simulink model "RB_KAIROS_BaseOnly"  (R2020b)
settings: Solver=ode4  StartTime=0.0  StopTime=t_end  FixedStep=Ts  RelTol=1e-3
values from neighbouring files (symbols this model uses):
  am = 0.3    [RB_KAIROS_ImpControl_OpSpace_BaseOnly.m]
  am_r = 0.3    [RB_KAIROS_ImpControl_OpSpace_BaseOnly.m]
  Jv = [1 0 0; 0 1 0; 0 0 0; 0 0 0; 0 0 0; 0 0 1;]    [RB_KAIROS_ImpControl_OpSpace_BaseOnly.m]
  Kc = diag(5*[1000,1000,0,0,0,1000])    [RB_KAIROS_ImpControl_OpSpace_BaseOnly.m]
  model_sample_time = 0.001    [RB_KAIROS_ImpControl_OpSpace_BaseOnly.m]
  q_dot_0 = zeros(10,1)    [RB_KAIROS_ImpControl_OpSpace_BaseOnly.m]
  T_i = T_W_V    [RB_KAIROS_ImpControl_OpSpace_BaseOnly.m]
  tau_ext = [0 0 0]    [RB_KAIROS_ImpControl_OpSpace_BaseOnly.m]
  v_SMU = 10    [RB_KAIROS_ImpControl_OpSpace_BaseOnly.m]
  vm = 0.6    [RB_KAIROS_ImpControl_OpSpace_BaseOnly.m]
  vm_r = 0.6    [RB_KAIROS_ImpControl_OpSpace_BaseOnly.m]
undefined symbols (not defined in the file or in its folder): DiscIntNeverNeededParam, magnitude, q_0, T_f
libraries: simulink x4, utils x4, transformations_lib x1
(part 15 of 16)

== matlab function RB_KAIROS_BaseOnly/Trajectory Generator/move2pose/Cartesian_ipol2/translation/Embedded MATLAB Function1 ==
  data: t input; qd output; s0 input; v0 input; sf input; vd input; am input; Tm input; T_scale input; interpoly input; time_step input; start_opt input; rethink_point input; start_lvl input; stop_lvl input; v_smu input; vm input; dqd output; ddqd output; ipol_finished output; opti_break output; T_est output
function [qd,dqd,ddqd, ipol_finished, opti_break, T_est] = calc_qd(t,s0,v0,sf,vd,am,Tm,T_scale,interpoly,time_step,start_opt,rethink_point,start_lvl,stop_lvl,v_smu,vm)
%%% This function decides which version to call; Or when/if a rethink is
%%% done.
% 0 = internship version (only with minor bugfixes)
% 1 = start with half the velocity, then rethink, then linear part and
% rest is the original full half
% 2 = start with full half rethink, again full half (Mazins way)
% 3 = general solution, heading to vm always (best option)
% 4 = general solution, heading to v_smu if going down (Mazins way)

qd = 0;
dqd = 0;
ddqd = 0;
ipol_finished = 0;
opti_break = 0;
T_est = 0;
switch rethink_point
    case 0
        [qd,dqd,ddqd, ipol_finished] = calc_qd_f(t,s0,v0,sf,vd,am,T_scale,interpoly,time_step);
    case 1
        [qd,dqd,ddqd, ipol_finished, opti_break, T_est] = calc_qd_hlf(t,s0,v0,sf,vd,am,Tm,T_scale,interpoly,time_step,start_opt);
    case 2
        [qd,dqd,ddqd, ipol_finished, opti_break, T_est] = calc_qd_ff(t,s0,v0,sf,vd,am,Tm,T_scale,interpoly,time_step,start_opt);
    case 3
        [qd,dqd,ddqd, ipol_finished, opti_break, T_est] = calc_qd_g(t,s0,v0,sf,vd,am,Tm,T_scale,interpoly,time_step,start_opt,start_lvl,stop_lvl,v_smu,vm,rethink_point);
    case 4
        [qd,dqd,ddqd, ipol_finished, opti_break, T_est] = calc_qd_g(t,s0,v0,sf,vd,am,Tm,T_scale,interpoly,time_step,start_opt,start_lvl,stop_lvl,v_smu,vm,rethink_point);
    otherwise
        error('Unknown rethink_point');       %rest
end


end

function [qd,dqd,ddqd, ipol_finished, opti_break, T_est] = calc_qd_g(t,s0,v0,sf,vd,am,Tm,T_scale,interpoly,time_step,start_opt,start_lvl,stop_lvl,v_smu,vm,rethink_point)
% This function calculates a one dimensional movement with a trapezodial 
% signal for velocity over time. Additionally it is able to adapt to shifts
% in the maximum allowed velocity.
%
% This is the most general solution so far. It accelerates till am and then
% it stays on this level till it has to decelerate again to reach the new
% velocity level. The velocity level could be updated in any timestep.
%
% Inputs:
% t         current runtime
% s0        start value for motion in position
% v0        start value for motion in velocity
% sf        final value for motion in position
% vd        desired velocity
% am        maximum allowed acceleration
% Tm        Maximum time left for adaption
% T_scale   Scaling factor for duration of adaption
% interpoly Which interpolation to use
% time_step Duration of one time step
% start_opt Options for prevent errors at start and end; see below
% start_lvl percentage for delta_v_start: [0;1[ (Do not set to near to one!)
% stop_lvl  percentage for delta_v_stop: [0;1[ (Do not set to near to one!)
% v_smu     Real v_smu
% vm        maximum allowed velocity
% rethink_point
%           choose on which velocity the percentage is used
%
% Outputs:
% qd        disered position at current time
% dqd       disered velocity at current time
% ddqd      disered acceleration at current time
% ipol_finished 
%           motion is finished
% opti_break
%           Trigger for optimal breaking; is set to 1 if Tm<T_est
% T_est     Current estimate of the duration of the adaption motion

% Start / end options:
% 0 = Do nothing; Not recommanded, because of unstable behaviour, since start phase not programmed
% 1 = Delay till adaption possible (Best option I think)
% 2 = Delay till adaption possible and vd is updated


% In general variables with ..._1 belong to previous runs of the code and
% variables with numbers at the end belong to the corresponding phase. 
% Phase 1 is the start of an adaption motion. On this phase the
% acceleration is increased to am. In phase 2 the acceleration is constant
% on level am, which means that the velocity is linear. The decrease of the
% acceleration to zero again is called phase 3.
% A single i in the name of a varibale, means an inital value of something
% and the same holds for f for final value. m is maximum, d is desired, c
% is current.
% q is a vector with (position,velocity,acceleration). Small t is a absolut
% time, whereas capital T is a time duration.


T_est = 0; %init Duration estimate
v_eps = 1e-4; %lowest velocity difference an adaption starts

% Code can not stop the motion => vd must be >0 (because of t_shift calc)
if vd<v_eps
    vd=v_eps;
end

%% Initialize persistent variables for adaption motion
persistent vd_1 adpt adpt_run phase restart ti1 qi1 qf1 T1 t_shift t_shift3 t_shift_1 T2 T3 ti2 parameter2 ti3 qf3 qi3 delta_q3 adpt_blanking adpt_blanking_end opti_break_mem v_delta_stop v_delta_start
if isempty(vd_1)
    vd_1 = vd;       %remembers the max velocity from last run
end
if isempty(adpt)
    adpt = false;   %stores if an adaption motion is activated
end
if isempty(adpt_run)
    adpt_run = false;   %stores if an adaption motion is activated
end
if isempty(phase)
    phase = 0;         %phase of adaption
end
if isempty(restart)
    restart = -1;         %At end of phase 3 the current velocity must be stored and restarts an adpation process
end
if isempty(t_shift)
    t_shift = 0;    %Time distance with which the current reference motion is shifted
end
if isempty(t_shift_1)
    t_shift_1 = 0;    %Time distance with which the old reference motion was shifted
end
if isempty(ti1)
    ti1 = 0;         %Initial time step for adaption motion
end
if isempty(T1)
    T1 = 0;          %Duration of complete adaption motion; tf = ti+T
end
if isempty(qi1)
    qi1 = zeros(3,1);%Initial values (pos,vel,acc) for adaption motion
end
if isempty(qf1)
    qf1 = zeros(3,1);%Final values (pos,vel,acc) for adaption motion
end
if isempty(ti2) 
    ti2 = 0;         %Initial time for linear part  (phase 2)
end
if isempty(T2)
    T2 = 0;         %Exact duration of phase 2
end
if isempty(parameter2)
    parameter2 = zeros(3,1);         %Parameter of linear part / phase 2: 0.5*p(3)*t^2 + p(2)*t + p(1)
end
if isempty(ti3)
    ti3 = 0;         %Initial time for phase 3
end
if isempty(T3)
    T3 = 0;         %Duration of phase 3 (But seen from start in the past; so actually it is T/2)
end
if isempty(qi3)
    qi3 = zeros(3,1); %Initial values (pos,vel,acc) for phase 3
end
if isempty(qf3)
    qf3 = zeros(3,1); %Final values (pos,vel,acc) for phase 3
end
if isempty(t_shift3)
    t_shift3 = 0;    %Time distance with which the updated reference motion is shifted (phase 3)
end
if isempty(delta_q3)
    delta_q3 = 0;         %shift of position in phase 3
end
if isempty(adpt_blanking)
    adpt_blanking = -1;         %memory of current vd for startopt 2
end
if isempty(adpt_blanking_end)
    adpt_blanking_end = -1;         %memory of last vd before adaption while deceleration phase
end
if isempty(opti_break_mem)
    opti_break_mem = 0;         %memory of opti break; (holds trigger while adaption)
end
if isempty(v_delta_start)
    v_delta_start = 0;         %delta of velocity which the start of an adaption needs
end
if isempty(v_delta_stop)
    v_delta_stop = 0;         %delta of velocity which the stop of an adaption needs
end

%% This If runs only for one timestep!!!
% If current desired velocity is unequal to old one 
% Not directly at the beginning
% Dont start new while a adaption is still running, to prevent reset of
%   initial values
% Or restart is requested at end of last adaption
% And do nothing anymore if last adaption has collided with end 
if adpt_blanking_end==-1 && adpt==false && (...
        (vd~=vd_1 && t>time_step)...
        || restart>=0 )
            
    
    if restart==vd %This if prevents a adaption if restart was set to the current vd (only possible with startoptions or low velocity)
        adpt = false;
        phase = 0;
        restart = -1;
        adpt_blanking = -1;
        
    % This if prevents adaptions if the difference in the desired velocity
    % is below the threshold v_eps. To save the current velocity the
    % restart variable is used again. This also means that if the vd is
    % changing with a rate lower than the threshold, it is neccessary to
    % also compare the current velocity (in restart) and the current
    % desired velocity. If these two are more than the threshold it is
    % possible to adapt with the minimum adaption function.
    elseif (restart==-1 && abs(vd-vd_1)<v_eps) ||...
           (restart>=0  && abs(vd-vd_1)<v_eps && abs(vd-restart)<v_eps)
        adpt = false; 
        phase = 0;
        if restart == -1 %For preventing a small error, because the vd has changed, while the non-adaption calculation
           restart = vd_1; 
        end
        
    % If no reasons so far to prevent adaption, start the adaption:
    else
        adpt = true;          % Activate adaption 
        phase = 1;            % Start with phase 1
        t_shift_1 = t_shift;  % Store old time shift if adaption is reseted because of start/end phase of mogen 
        ti1 = t;              % Set initial timestep to current step  

        %%% inital set of position, velo, acceleration for adaption motion 
        % is the same as the old mogen would do (t_shift is not updated at
        % this time!)
        if restart>=0 %If restart is requested, the current velocity is stored in the restart variable
            [qi1, ~] = interpolator(ti1+t_shift, compute_traj_parameters(s0, v0, sf, restart, am));
        else
            [qi1, ~] = interpolator(ti1+t_shift, compute_traj_parameters(s0, v0, sf, vd_1, am));
        end

        %%% Calc basic velocity levels
        vc = qi1(2);    % current velocity = restart velocity or vd_1
        vf = vd;        % v_final is current global final velocity
        v_heading = vf; % v_heading the velocity level the program is looking to, while calculating the v_deltas

        %For making sure that it is heading to v_smu always, while going down (Mazins way)
        if rethink_point == 4 && vd<vc
            v_heading = v_smu; 
        end

        % velocity deltas at begin and end of adaption: 
        % mind the signs!!
        v_delta_start = ((v_heading-vc)*(1-start_lvl))/2;
        v_delta_stop  = ((vc-v_heading)*(1-stop_lvl))/2;

        %%% Calculation of Phase 1 and basic parameters

        % computes the time shift for shifting the new motion to the end
        % point of the old motion. So at which time the new motion has
        % the same qd? Then calculate the time distance to the inital
        % time of the change in velocities
        % t_shift < 0 if new motion is faster (vd>vd_1)
        % t_shift > 0 if new motion is slower (vd<vd_1)
        % interpolator_1 is the inverse function of interpolator!
        vf1 = vc+2*v_delta_start; %This is the final velocity of the start / phase 1
        t_shift_inv = interpolator_1(qi1(1), compute_traj_parameters(s0, v0, sf, vf1, am));
        t_shift = t_shift_inv - ti1 ;

        % Calculate duration of adaption in phase 1
        if interpoly==0 % if interpolation is zero no adaption is requested, but the t_shift has to be calculated anyway
            adpt = false;
            phase = 0;
            restart = -1;
            adpt_blanking = -1;
        else
            T1 = T_calc(vc,vf1,am,T_scale,interpoly); 
            %T1 = T_calc_a_scale(vc,vf1,vm,v_eps,am,time_step,T_scale,interpoly); 
        end

        % The additional shift for adaption motion is dependent on the
        % difference in the velocities. See report for details.
        t_shift = t_shift+(T1/2)*((vc/vf1)-1);

        % Calculate final values for adaption motion. Which are reached
        % at inital time plus duration of adaption and new time shift
        [qf1, ~] = interpolator(ti1+t_shift+T1, compute_traj_parameters(s0, v0, sf, vf1, am));

        %%% Parameters for Phase 2 / linear part

        ti2 = ti1+T1/2; % initial time of linear part

        % calculate state of phase 1 at start of phase 2, which are the
        % parameters of phase 2, since phase 2 has its time orgin at the
        % same point.
        parameter2 = adpt_fct(ti2,ti1,T1,qi1,qf1,vd,am,interpoly); 

        %%% Check if errors occured so far due to acc/dec phase
        % check start phase
        if qi1(3)>0 || qf1(3)>0 || t_shift_inv == 0 %If interpolator in acc phase or invers interpolator is not jet available
            if start_opt == 1 
                adpt = false; 
                phase = 0;
                t_shift = t_shift_1; %Reset calculated t_shift
                if restart == -1 % For delaying the start of the adaption, the restart is used and set to the current value, if not done already
                   restart = vd_1; 
                end
            elseif start_opt == 2 % For delay and wait on update, the restart is set and ...
                adpt = false;
                phase = 0;
                t_shift = t_shift_1; %Reset calculated t_shift
                adpt_blanking = vd; % ... the adpt_blanking variable is set to the current new velocity.
                if restart == -1
                   restart = vd_1; 
                end
            end
        elseif start_opt>0 && (qi1(3)<0 || qf1(3)<0 || t_shift_inv == -1 ) %If interpolator in dec phase or invers interpolator is no more available
            % if adaption is colliding with the decelaration phase of mogen,
            % the adpt_blanking_end variable is used, which prevents all
            % atempts for an adaption
            if restart>=0
                adpt_blanking_end = restart; %If the adaption was triggerd with restart, the current velocity is there too
            else
                adpt_blanking_end = vd_1;
            end
            adpt = false; 
            phase = 0;
            t_shift = t_shift_1;
            restart = -1;
            adpt_blanking = -1;
        elseif adpt_blanking == vd % Only for startopt==2: If adaption would be possible, the code now waites for an update of vd.
            adpt = false;
            phase = 0;
            t_shift = t_shift_1;
        end  
    end
end

%% Update function; runs always in phase 1 and phase 2 to update duration and check final levels
if adpt == true && (phase == 1 || phase == 2)
    
    %%% First decide to which velocity the program should go. This is
    %%% necessesary since the current vd could be higher than the velocity
    %%% level wich could be reached with an imdiate introduction of phase
    %%% 3. This nearest velocity level which can currently be reached is
    %%% called v_near and calculated first   
    
    % evaluate linear part at last timestep
    t2 = t-ti2-time_step; 
    q2 = zeros(3,1); 
    q2(1) = 0.5*parameter2(3)*t2^2+parameter2(2)*t2+parameter2(1);
    q2(2) = parameter2(3)*t2+parameter2(2);
    q2(3) = parameter2(3);

    % Calculate nearest velocity v_near
    if phase == 1
        % in phase 1 it is the start velocity plus both deltas, without
        % linear part
        v_near = qi1(2)+v_delta_start-v_delta_stop; %mind the signs!!!
    else
        % while linear part it is the current velocity level plus what is
        % needed to stop adaption.
        v_near = q2(2)-v_delta_stop; %mind the signs!!!
    end
    
    % this is now the decision to which velocity the update should go to
    if qi1(2)>qf1(2) && vd>=v_near
        vd_up = v_near;
    elseif qi1(2)<qf1(2) && vd<=v_near
        vd_up = v_near;
    else
        % check if it is still possible to reach at least v_near in the
        % next step (called v_near_p1). Because if the vd changes in the
        % next step so that it is no more possible to reach vd, the
        % adaption has to stop at v_near_p1 in the next step and therefore
        % v_near_p1 has to be reachable. If even this is not possible, then
        % stop now at v_near.

        % evaluate linear part at current timestep
        t2 = t-ti2; 
        q2 = zeros(3,1); 
        q2(1) = 0.5*parameter2(3)*t2^2+parameter2(2)*t2+parameter2(1);
        q2(2) = parameter2(3)*t2+parameter2(2);
        q2(3) = parameter2(3);

        % Calculate nearest velocity v_near_p1
        if phase == 1
            % in phase 1 it is the start velocity plus both deltas, without
            % linear part
            v_near_p1 = qi1(2)+v_delta_start-v_delta_stop; %mind the signs!!!
        else
            % while linear part it is the current velocity level plus what is
            % needed to stop adaption.
            v_near_p1 = q2(2)-v_delta_stop; %mind the signs!!!
        end
        
        % Evaluate function at v_near_p1 for next time step
        [~,~,~,~,~,~,~,error_state_p1] = calc_g_update_fct(v_near_p1,v_delta_stop,qi1,ti2,parameter2,am,T_scale,interpoly,s0, v0, sf,start_opt,vm,v_eps,time_step);
        if start_opt >0 && error_state_p1==2 %If errors with dec phase
            vd_up = v_near;
        else        
            vd_up = vd;
        end
    end 
    
    [T2,T3,ti3,qi3,qf3,delta_q3,t_shift3,error_state] = calc_g_update_fct(vd_up,v_delta_stop,qi1,ti2,parameter2,am,T_scale,interpoly,s0, v0, sf,start_opt,vm,v_eps,time_step);
    
    if adpt_run==false
        %%% Check if adaption is possible before it actually has started; means check error_state
        if error_state==1 %If errors with acc phase
            if start_opt == 1 
                adpt = false; 
                phase = 0;
                t_shift = t_shift_1; %Reset calculated t_shift
                if restart == -1 % For delaying the start of the adaption, the restart is used and set to the current value, if not done already
                   restart = vd_1; 
                end
            elseif start_opt == 2 % For delay and wait on update, the restart is set and ...
                adpt = false;
                phase = 0;
                t_shift = t_shift_1; %Reset calculated t_shift
                adpt_blanking = vd; % ... the adpt_blanking variable is set to the current new velocity.
                if restart == -1
                   restart = vd_1; 
                end
            end
        elseif start_opt >0 && error_state==2 %If errors with dec phase
            % if adaption is colliding with the decelaration phase of mogen,
            % the adpt_blanking_end variable is used, which prevents all
            % atempts for an adaption
            if restart>=0
                adpt_blanking_end = restart; %If the adaption was triggerd with restart, the current velocity is there too
            else
                adpt_blanking_end = vd_1;
            end
            adpt = false; 
            phase = 0;
            t_shift = t_shift_1;
            restart = -1;
            adpt_blanking = -1;
        else % Triggered if adaption is possible and will start now
            % Reset variables
            restart = -1;
            adpt_blanking = -1;
        end 
    else
        % adaption is already running; means no problems possible at start 
        % points, but if current endpoint is colliding with deceleration
        % phase, take v_near to stop.
        if start_opt >0 && error_state==2 %If errors with dec phase
            [T2,T3,ti3,qi3,qf3,delta_q3,t_shift3,~] = calc_g_update_fct(v_near,v_delta_stop,qi1,ti2,parameter2,am,T_scale,interpoly,s0, v0, sf,start_opt,vm,v_eps,time_step);
        end
    end

end

%% This If runs only for one timestep!!!
% Phase 1 => Phase 2
if phase == 1 && t>=ti2 %End of phase 1
    phase = 2;
end

%% This If runs only for one timestep!!!
% Phase 2 => Phase 3
if phase == 2 && t>=ti3 %End of phase 2
    phase = 3;
    t_shift = t_shift3; %Activate new t_shift for phase 3
end

%% Here the actual motion is calculated
% Interpolates the values of pos,vel,acc (qv) with parameters and current time t 

if restart >=0
    [qdv, ipol_finished] = interpolator(t+t_shift, compute_traj_parameters(s0, v0, sf, restart, am));
elseif adpt_blanking_end >=0
    [qdv, ipol_finished] = interpolator(t+t_shift, compute_traj_parameters(s0, v0, sf, adpt_blanking_end, am));
else
    [qdv, ipol_finished] = interpolator(t+t_shift, compute_traj_parameters(s0, v0, sf, vd, am));
end  

%% If adaption motion needed
if adpt == true
    
    adpt_run = true;
    ipol_finished=0;%Prevent finish command from old interpolator
    % Calc adaption motion
    if phase == 1
        % opti_break
        T_est = (T1/2+T2+T3/2)-(t-ti1);
        if Tm<T_est
            opti_break_mem = 1; 
        end
        % accelerate till am
        qdv = adpt_fct(t,ti1,T1,qi1,qf1,vd,am,interpoly);
    elseif phase == 2
        % opti_break
        T_est = ((T2+T3/2)-(t-ti2));
        if Tm<T_est
            opti_break_mem = 1; 
        end
        % linear part
        t2 = t-ti2;
        qdv = zeros(3,1);
        qdv(1) = 0.5*parameter2(3)*t2^2+parameter2(2)*t2+parameter2(1);
        qdv(2) = parameter2(3)*t2+parameter2(2);
        qdv(3) = parameter2(3);
    elseif phase == 3
        %if time is equal than the finish time => adaption motion is complete
        %But it is aborted one timestep earlier, since the finish timestep
        %is already computed correctly by the standard interpolator.
        if t>=ti3+T3/2-1*time_step  
            adpt=false;     %If adaption finished => reset
            phase = 0;
            adpt_run = false;
            opti_break_mem = 0; % also reset opti break
            % Calculate finish time_step here because vd could be not equal
            % to final reached velocity level
            [qdv, ipol_finished] = interpolator(t+t_shift, compute_traj_parameters(s0, v0, sf, qf3(2), am)); 
            if vd~=qf3(2)  %If adaption is finished, but the vd value has changed again => restart from current velocity on
                restart = qf3(2);
            else
                restart = -1;
            end            
        else
            % opti_break
            T_est = T3/2-(t-ti3);
            if Tm<T_est
                opti_break_mem = 1; 
            end
        
            % Adaption to vd velocity
            delta_q_vec = zeros(3,1);
            delta_q_vec(1) = delta_q3; %Build delta_q vector
            tx = -T3/2;
            % Evaluate adaption function, shift with tx in time ...
            qdv = adpt_fct(t,ti3+tx,T3,qi3,qf3,vd,am,interpoly) - delta_q_vec;
        end 
        
    end

end

%% Set output
if sf == s0          % No motion needed if start = end 
    qd = s0;         % => set initial values
    dqd = v0;
    ddqd = 0;  
else     
    qd = qdv(1);     % set output
    dqd = qdv(2);
    ddqd = qdv(3);        
end
opti_break = opti_break_mem; %set opti break output (Simulink cannot use persistent variable as output)
vd_1 = vd;  %remember current max velocity

end

function [qd,dqd,ddqd, ipol_finished, opti_break, T_est] = calc_qd_hlf(t,s0,v0,sf,vm,am,Tm,T_scale,interpoly,time_step,start_opt)
% This function calculates a one dimensional movement with a trapezodial 
% signal for velocity over time. Additionally it is able to adapt to shifts
% in the maximum allowed velocity.
%
% This is the more adaptive version which rethinks about the target
% velocity after the maximum acceleration is reached. And also it is
% allowed to change the velocity reference while an adaption is running.
%
% Inputs:
% t         current runtime
% s0        start value for motion in position
% v0        start value for motion in velocity
% sf        final value for motion in position
% vm        maximum allowed velocity
% am        maximum allowed acceleration
% Tm        Maximum time left for adaption
% T_scale   Scaling factor for duration of adaption
% interpoly Which interpolation to use
% time_step Duration of one time step
% start_opt Options for prevent errors at start and end; see below
%
% Outputs:
% qd        disered position at current time
% dqd       disered velocity at current time
% ddqd      disered acceleration at current time
% ipol_finished 
%           motion is finished
% opti_break
%           Trigger for optimal breaking; is set to 1 if Tm<T_est
% T_est     Current estimate of the duration of the adaption motion

% Start / end options:
% 0 = Do nothing; Not recommanded, because of unstable behaviour, since start phase not programmed
% 1 = Delay till adaption possible (Best option I think)
% 2 = Delay till adaption possible and vm is updated

%% Initialize persistent variables for adaption motion
persistent vm1 adpt phase restart ti qi qf T t_shift t_shift_up t_shift_1 T_lin T_up vf ti_lin shift slope c ti_up qf_up qi_up delta_q adpt_blanking adpt_blanking_end opti_break_mem
if isempty(vm1)
    vm1 = vm;       %remembers the max velocity from last run
end
if isempty(adpt)
    adpt = false;   %stores if an adaption motion is activated
end
if isempty(phase)
    phase = 0;         %phase of adaption
end
if isempty(restart)
    restart = -1;         %At end of phase 4 the current velocity must be stored and restarts an adpation process
end
if isempty(ti)
    ti = 0;         %Initial time step for adaption motion
end
if isempty(qi)
    qi = zeros(3,1);%Initial values (pos,vel,acc) for adaption motion
end
if isempty(qf)
    qf = zeros(3,1);%Final values (pos,vel,acc) for adaption motion
end
if isempty(T)
    T = 0;          %Duration of complete adaption motion; tf = ti+T
end
if isempty(t_shift)
    t_shift = 0;    %Time distance with which the current reference motion is shifted
end
if isempty(t_shift_up)
    t_shift_up = 0;    %Time distance with which the updated reference motion is shifted
end
if isempty(t_shift_1)
    t_shift_1 = 0;    %Time distance with which the old reference motion was shifted
end
if isempty(T_lin)
    T_lin = 0;         %Exact duration of phase 2
end
if isempty(T_up)
    T_up = 0;         %Duration of phase 3 (But seen from start in the past; so actually it is T/2)
end
if isempty(vf)
    vf = 0;         %global final velocity at start of adaption motion
end
if isempty(ti_lin) 
    ti_lin = 0;         %Initial time for linear part  (phase 2)
end
if isempty(shift)
    shift = 0;         %shift of linear part (phase 2)
end
if isempty(slope)
    slope = 0;         %slope of linear part (phase 2)
end
if isempty(c)
    c = 0;         %integration const of linear part (phase 2)
end
if isempty(ti_up)
    ti_up = 0;         %Initial time for phase 3
end
if isempty(qf_up)
    qf_up = zeros(3,1); %Final values (pos,vel,acc) for phase 3
end
if isempty(qi_up)
    qi_up = zeros(3,1); %Initial values (pos,vel,acc) for phase 3
end
if isempty(delta_q)
    delta_q = 0;         %shift of position in phase 3
end
if isempty(adpt_blanking)
    adpt_blanking = -1;         %memory of current vm for startopt 2
end
if isempty(adpt_blanking_end)
    adpt_blanking_end = -1;         %memory of last vm before adaption while deceleration phase
end
if isempty(opti_break_mem)
    opti_break_mem = 0;         %memory of opti break; (holds trigger while adaption)
end
T_est = 0; %init

%% This If runs only for one timestep!!!
% If current max velocity is unequal to old one 
% Not directly at the beginning
% Dont start new while a adaption is still running, to prevent reset of
%   initial values
% Or restart is requested at end of last adaption
if abs(vm-vm1)>1e-3 && t>time_step && adpt==false ...
        || restart>=0 && adpt==false  
    adpt = true;          % Activate adaption         
    ti = t;               % Set initial timestep to current step  
    
    %init some variables for simulink
    t_inv = 0; 
    t_inv_f = 0;
    v_current = 0;
    v_goal = 0;
    
    if restart==vm %This if prevents a adaption if restart was set to the current vm (only with startoptions)
        adpt = false;
        ti = 0;
        restart = -1;
        adpt_blanking = -1;
    else
        %%% inital set of position, velo, acceleration for adaption motion 
        % is the same as the old mogen would do (t_shift is not updated at
        % this time!)
        if restart>=0 %If restart is requested, the current velocity is stored in the restart variable
            [qi, ~] = interpolator(ti+t_shift, compute_traj_parameters(s0, v0, sf, restart, am));
        else
            [qi, ~] = interpolator(ti+t_shift, compute_traj_parameters(s0, v0, sf, vm1, am));
        end

        vf = vm; % vf is current global final velocity
        v_current = qi(2); % current velocity = restart velocity or vm1
        v_goal = 0.5*(vf+v_current); %intermediate goal velocity

        % Check if adaption is possible; Therefore the inverse functions
        % must be available.
        t_inv = interpolator_1(qi(1), compute_traj_parameters(s0, v0, sf, v_goal, am)) ;
        t_inv_f = interpolator_1(qi(1), compute_traj_parameters(s0, v0, sf, vf, am));
        % If they return zero an adaption is not possible since start phase
        % is active; 
        % Another reason for no adaption is that the current acceleration 
        % is not zero.
        if t_inv == 0 || t_inv_f == 0 || qi(3)>0
            if start_opt == 1 % For delaying the start, the restart is used and set to the current value, if not done already
                adpt = false; 
                ti = 0;
                if restart == -1
                   restart = vm1; 
                end
            elseif start_opt == 2 % For delay and wait on update, the restart is set and ...
                adpt = false;
                ti = 0;
                adpt_blanking = vm; % ... the adpt_blanking variable is set to the current new velocity.
                if restart == -1
                   restart = vm1; 
                end
            end
        end  
    end
    
    if start_opt >0 && qi(3)<0
        adpt_blanking_end = vm1;
        adpt = false; 
        ti = 0;
        restart = -1;
        adpt_blanking = -1;
    end
    
    if adpt_blanking == vm % Only for startopt==2: If adaption would be possible, the code now waites for an update of vm.
        adpt = false;
        ti = 0;
    end
    
    if adpt == true
        % Really start with an adaption now!
        phase = 1;            % Start with phase 1

        % Store old time shift for later calculation of virtual shift
        t_shift_1 = t_shift;

        %%% Calculation of Phase 4 and basic parameters
        
        % computes the time shift for shifting the new motion to the end
        % point of the old motion. So at which time the new motion has
        % the same qd? Then calculate the time distance to the inital
        % time of the change in velocities
        % t_shift < 0 if new motion is faster (vm>vm1)
        % t_shift > 0 if new motion is slower (vm<vm1)
        % interpolator_1 is the inverse function of interpolator!
        t_shift = t_inv - ti ;

        % Calculate duration of adaption
        if interpoly==0 
            T = 0;
            adpt = false;
            phase = 0;
        else
            T = T_calc(v_current,v_goal,am,T_scale,interpoly)*2; %*2 to fit to Mazins way
        end

        % The additional shift for adaption motion is dependent on the
        % difference in the velocities. See report for details.
        t_shift = t_shift+(T/4)*((v_current/v_goal)-1);

        % Calculate final values for adaption motion. Which are reached
        % at inital time plus duration of adaption and new time shift
        [qf, ~] = interpolator(ti+t_shift+T/2, compute_traj_parameters(s0, v0, sf, v_goal, am));

        %%% Parameters for Phase 2 / linear part
        
        ti_lin = ti+T/4; % initial time of linear part
        
        % calculate current state with adaption from phase 1
        q_current = adpt_fct(ti_lin,ti,T/2,qi,qf,vm,am,interpoly);        
        
        % Calculate parameters for linear part in phase 2
        slope = q_current(3);   %slope of lin part is acceleration of current state
        shift = q_current(2);   %shift of lin part is velocity of current state
        c = q_current(1);       %Position constant is position of current state
        T_lin = ((0.5*(qi(2)+vf)-shift)/slope);% Exact Duration of linear part

        
        %%% Parameters for Phase 3
        ti_up = ti_lin+T_lin; % initial time for phase 3
    
        % calculate what linear part would do now = final value of phase 2
        dt = T_lin;
        qf_lin = zeros(3,1); %final value of phase 2
        qf_lin(1) = 0.5*slope*dt^2+shift*dt+c;
        qf_lin(2) = slope*dt+shift;
        qf_lin(3) = slope;

        T_up = T; % This not directly the duration of phase 3, because of the virtual part in the past
        qi_up = qi; % The final adaption motion starts at the same point as the first
        tx = (T/4)-T_lin; %exact time shift resulting from linear part

        % Calculate a time shift for the interpolator, as if the vf was
        % triggered right at the start (ti)
        t_shift_inter = t_inv_f - ti ;
        t_shift_inter = t_shift_inter+(T/2)*((qi_up(2)/vf)-1);

        % Also calculate final values, as if the vf was triggered right at the
        % start.
        [qf_up, ~] = interpolator(ti+t_shift_inter+T, compute_traj_parameters(s0, v0, sf, vf, am));

        % From now on this initial and final values are used in the adaption
        % function for the phase 3. This function is now also shifted in time
        % with the tx value, so starting time is ti-tx.

        % Next step is to evaluate this function at ti_up, which is the current
        % time, to get the position is function would do.
        q_dir_adpt = adpt_fct(ti_up,ti-tx,T_up,qi_up,qf_up,vm,am,interpoly);
        % The difference of the adaption motion position and current position
        % of the final values of the linear part, is now used to shift the
        % adaption also in position level to the current values.
        delta_q = q_dir_adpt(1) - qf_lin(1);
        delta_q_vec = zeros(3,1);
        delta_q_vec(1) = delta_q;

        % Next step is to calculate the real final values, which are the same
        % as the direct ones in velocity and acceleration level. But for
        % position level one needs to respect the delta_q shift.
        qf_real = qf_up - delta_q_vec;

        % To fit the interploator function at this final values again, a new
        % time shift is calculated 
        t_shift_up = interpolator_1(qf_real(1), compute_traj_parameters(s0, v0, sf, vf, am)) - (ti+T_up-tx) ;

        % test line; Should be all ==0
        %test_diff = q_dir_adpt-delta_q_vec -qf_lin;

        
        %%% blanking for deceleration phase
        if start_opt >0 && (qf(3)~=0 || qf_up(3)~=0)
            if restart>=0
                adpt_blanking_end = restart;
            else
                adpt_blanking_end = vm1;
            end
            adpt = false;
            phase = 0;
            t_shift = t_shift_1;
        end
        
        % Reset variables
        restart = -1;
        adpt_blanking = -1;
        
    end
end
    
%% This If runs only for one timestep!!!
% Rethink?! Phase 1 => Phase 2
if phase == 1 && t>=ti_lin %End of phase 1
    if qi(2)<vf && vm<=qf(2) % If human stops or goes away meanwhile
        phase = 4;
    elseif qi(2)>vf && vm>=qf(2) % If human stops or goes away meanwhile
        phase = 4;
    else
        phase = 2;
    end 
end

%% This If runs only for one timestep!!!
% Phase 2 => Phase 3
if phase == 2 && t>=ti_up %End of phase 2
    phase = 3;
    t_shift = t_shift_up;
end

%% Here the actual motion is calculated
% Interpolates the values of pos,vel,acc (qv) with parameters and current time t 

if restart >=0
    [qdv, ipol_finished] = interpolator(t+t_shift, compute_traj_parameters(s0, v0, sf, restart, am));
elseif adpt_blanking_end >=0
    [qdv, ipol_finished] = interpolator(t+t_shift, compute_traj_parameters(s0, v0, sf, adpt_blanking_end, am));
else
    [qdv, ipol_finished] = interpolator(t+t_shift, compute_traj_parameters(s0, v0, sf, vm, am));
end  

%% If adaption motion needed
if adpt == true
    
    %%% Calc adaption motion
    ipol_finished=0;%Prevent finish command from old interpolator
    if phase == 1
        %%% opti_break
        T_est = ((0.75*T+T_lin)-(t-ti));
        if Tm<T_est
            opti_break_mem = 1; 
        end
        % accelerate till am
        qdv = adpt_fct(t,ti,T/2,qi,qf,vm,am,interpoly);
    elseif phase == 2
        %%% opti_break
        T_est = ((0.5*T+T_lin)-(t-ti_lin));
        if Tm<T_est
            opti_break_mem = 1; 
        end
        % linear part
        qdv = zeros(3,1);
        dt = t-ti_lin;
        qdv(1) = 0.5*slope*dt^2+shift*dt+c;
        qdv(2) = slope*dt+shift;
        qdv(3) = slope;
    elseif phase == 3
        % decelerate to 0 and reach vf
        
        tx = (T/4)-T_lin; %exact time shift of linear part (again)
        %if time is equal than the finish time => adaption motion is complete
        %But it is aborted one timestep earlier, since the finish timestep
        %is already computed correctly by the standard interpolator.
        if t>=(ti-tx+T_up-1*time_step) 
            adpt=false;     %If adaption finished => reset
            phase = 0;
            opti_break_mem = 0; 
            % Calculate finish time_step
            [qdv, ipol_finished] = interpolator(t+t_shift, compute_traj_parameters(s0, v0, sf, vf, am));
            if vm~=vf  %If adaption is finished, but the vm value has changed again => restart from current velocity on
                restart = vf;
            else
                restart = -1;
            end
        else
            %%% opti_break
            T_est = ((0.5*T)-(t-ti_up));
            if Tm<T_est
                opti_break_mem = 1; 
            end
        
            delta_q_vec = zeros(3,1);
            delta_q_vec(1) = delta_q; %Build delta_q vector
            % Evaluate adaption function, shift with tx in time and with shift delta_q in position level
            qdv = adpt_fct(t,ti-tx,T_up,qi_up,qf_up,vm,am,interpoly) - delta_q_vec;
        end
        
    elseif phase == 4
        %if time is equal than the finish time => adaption motion is complete
        %But it is aborted one timestep earlier, since the finish timestep
        %is already computed correctly by the standard interpolator.
        if t>=(ti+T/2-1*time_step)  
            adpt=false;     %If adaption finished => reset
            phase = 0;
            opti_break_mem = 0; 
            restart = qf(2); %Imidiately Restart with the current velocity
            % Calculate finish time_step
            [qdv, ipol_finished] = interpolator(t+t_shift, compute_traj_parameters(s0, v0, sf, qf(2), am));
            
        else
            %%% opti_break
            T_est = ((0.25*T)-(t-ti_lin));
            if Tm<T_est
                opti_break_mem = 1; 
            end
        
            % Adaption to intermediate velocity
            qdv = adpt_fct(t,ti,T/2,qi,qf,vm,am,interpoly); 
        end 
        
    end

end

%% Set output
if sf == s0          % No motion needed if start = end 
    qd = s0;         % => set initial values
    dqd = v0;
    ddqd = 0;  
else     
    qd = qdv(1);     % set output
    dqd = qdv(2);
    ddqd = qdv(3);        
end
opti_break = opti_break_mem;
vm1 = vm;  %remember current max velocity

end

function [qd,dqd,ddqd, ipol_finished, opti_break, T_est] = calc_qd_ff(t,s0,v0,sf,vm,am,Tm,T_scale,interpoly,time_step,start_opt)
% This function calculates a one dimensional movement with a trapezodial 
% signal for velocity over time. Additionally it is able to adapt to shifts
% in the maximum allowed velocity.
%
% This is the more adaptive version which rethinks about the target
% velocity after the maximum acceleration is reached. And also it is
% allowed to change the velocity reference while an adaption is running.
% The Rethink point is in this code at T/2.
%
% Inputs:
% t         current runtime
% s0        start value for motion in position
% v0        start value for motion in velocity
% sf        final value for motion in position
% vm        maximum allowed velocity
% am        maximum allowed acceleration
% Tm        Maximum time left for adaption
% T_scale   Scaling factor for duration of adaption
% interpoly Which interpolation to use
% time_step Duration of one time step
% start_opt Options for prevent errors at start and end; see below
%
% Outputs:
% qd        disered position at current time
% dqd       disered velocity at current time
% ddqd      disered acceleration at current time
% ipol_finished 
%           motion is finished
% opti_break
%           Trigger for optimal breaking; is set to 1 if Tm<T_est
% T_est     Current estimate of the duration of the adaption motion

% Start / end options:
% 0 = Do nothing; Not recommanded, because of unstable behaviour, since start phase not programmed
% 1 = Delay till adaption possible (Best option I think)
% 2 = Delay till adaption possible and vm is updated

%% Initialize persistent variables for adaption motion
persistent vm1 adpt phase restart ti qi qf T t_shift t_shift_up t_shift_1 T_lin T_up vf ti_lin shift slope c ti_up qf_up qi_up delta_q adpt_blanking adpt_blanking_end opti_break_mem
if isempty(vm1)
    vm1 = vm;       %remembers the max velocity from last run
end
if isempty(adpt)
    adpt = false;   %stores if an adaption motion is activated
end
if isempty(phase)
    phase = 0;         %phase of adaption
end
if isempty(restart)
    restart = -1;         %At end of phase 4 the current velocity must be stored and restarts an adpation process
end
if isempty(ti)
    ti = 0;         %Initial time step for adaption motion
end
if isempty(qi)
    qi = zeros(3,1);%Initial values (pos,vel,acc) for adaption motion
end
if isempty(qf)
    qf = zeros(3,1);%Final values (pos,vel,acc) for adaption motion
end
if isempty(T)
    T = 0;          %Duration of complete adaption motion; tf = ti+T
end
if isempty(t_shift)
    t_shift = 0;    %Time distance with which the current reference motion is shifted
end
if isempty(t_shift_up)
    t_shift_up = 0;    %Time distance with which the updated reference motion is shifted (phase 3)
end
if isempty(t_shift_1)
    t_shift_1 = 0;    %Time distance with which the old reference motion was shifted
end
if isempty(T_lin)
    T_lin = 0;         %Exact duration of phase 2
end
if isempty(T_up)
    T_up = 0;         %Duration of phase 3 (But seen from start in the past; so actually it is T/2)
end
if isempty(vf)
    vf = 0;         %global final velocity at start of adaption motion
end
if isempty(ti_lin) 
    ti_lin = 0;         %Initial time for linear part  (phase 2)
end
if isempty(shift)
    shift = 0;         %shift of linear part (phase 2)
end
if isempty(slope)
    slope = 0;         %slope of linear part (phase 2)
end
if isempty(c)
    c = 0;         %integration const of linear part (phase 2)
end
if isempty(ti_up)
    ti_up = 0;         %Initial time for phase 3
end
if isempty(qf_up)
    qf_up = zeros(3,1); %Final values (pos,vel,acc) for phase 3
end
if isempty(qi_up)
    qi_up = zeros(3,1); %Initial values (pos,vel,acc) for phase 3
end
if isempty(delta_q)
    delta_q = 0;         %shift of position in phase 3
end
if isempty(adpt_blanking)
    adpt_blanking = -1;         %memory of current vm for startopt 2
end
if isempty(adpt_blanking_end)
    adpt_blanking_end = -1;         %memory of last vm before adaption while deceleration phase
end
if isempty(opti_break_mem)
    opti_break_mem = 0;         %memory of opti break; (holds trigger while adaption)
end

T_est = 0; %init

%% This If runs only for one timestep!!!
% If current max velocity is unequal to old one 
% Not directly at the beginning
% Dont start new while a adaption is still running, to prevent reset of
%   initial values
% Or restart is requested at end of last adaption
if adpt_blanking_end==-1 && adpt==false && (...
        (abs(vm-vm1)>1e-3 && t>time_step)...
        || restart>=0 )
    adpt = true;          % Activate adaption         
    
    if restart==vm %This if prevents a adaption if restart was set to the current vm (only possible with startoptions)
        adpt = false;
        ti = 0;
        restart = -1;
        adpt_blanking = -1;
    end

    if adpt == true
        % Really start with an adaption now!
        ti = t;               % Set initial timestep to current step  
        phase = 1;            % Start with phase 1
        t_shift_1 = t_shift;  % Store old time shift for later calculation of virtual shift

        %%% inital set of position, velo, acceleration for adaption motion 
        % is the same as the old mogen would do (t_shift is not updated at
        % this time!)
        if restart>=0 %If restart is requested, the current velocity is stored in the restart variable
            [qi, ~] = interpolator(ti+t_shift, compute_traj_parameters(s0, v0, sf, restart, am));
        else
            [qi, ~] = interpolator(ti+t_shift, compute_traj_parameters(s0, v0, sf, vm1, am));
        end

        % Calc basic velocity levels
        v_current = qi(2); % current velocity = restart velocity or vm1
        vf = vm; % vf is current global final velocity
        v_inter_high = 0.25*(vf+3*v_current); %intermediate higher velocity
        v_inter = 0.5*(vf+v_current); %intermediate velocity
        v_inter_low = 0.25*(3*vf+v_current); %intermediate lower velocity

        %%% Calculation of Phase 1, 2 and basic parameters
        
        % computes the time shift for shifting the new motion to the end
        % point of the old motion. So at which time the new motion has
        % the same qd? Then calculate the time distance to the inital
        % time of the change in velocities
        % t_shift < 0 if new motion is faster (vm>vm1)
        % t_shift > 0 if new motion is slower (vm<vm1)
        % interpolator_1 is the inverse function of interpolator!
        t_inv = interpolator_1(qi(1), compute_traj_parameters(s0, v0, sf, vf, am)) ;
        t_shift = t_inv - ti ;

        % Calculate duration of adaption
        if interpoly==0 
            T = 0;
            adpt = false;
            phase = 0;
        else
            T = T_calc(v_current,vf,am,T_scale,interpoly); 
        end

        % The additional shift for adaption motion is dependent on the
        % difference in the velocities. See report for details.
        t_shift = t_shift+(T/2)*((v_current/vf)-1);

        % Calculate final values for adaption motion. Which are reached
        % at inital time plus duration of adaption and new time shift
        [qf, ~] = interpolator(ti+t_shift+T, compute_traj_parameters(s0, v0, sf, vf, am));
        
        %%% Parameters for Phase 3 (=update)
        ti_up = ti + T/2; % initial time for phase 3
    
        % calculate what phase 1 would do now = final value of phase 1
        qf_1 = adpt_fct(ti_up,ti,T,qi,qf,vm,am,interpoly);

        qi_up = [qi(1);v_inter_high;0]; %virtual starting point of phase 3; position wrong, but velocity correct
        T_up = T/2; % This not directly the duration of phase 3, because of the virtual part in the past
        tx = T/4; %exact time shift 

        % Calculate a time shift for the interpolator, from qi_up on
        t_inv_up = interpolator_1(qi_up(1), compute_traj_parameters(s0, v0, sf, v_inter_low, am));
        t_shift_inter = t_inv_up - (ti+tx);
        t_shift_inter = t_shift_inter+(T_up/2)*((qi_up(2)/v_inter_low)-1);

        % Also calculate final values
        [qf_up, ~] = interpolator(ti+tx+t_shift_inter+T_up, compute_traj_parameters(s0, v0, sf, v_inter_low, am));

        % From now on this initial and final values are used in the adaption
        % function for the phase 3. This function is now also shifted in time
        % with the tx value, so starting time is ti+tx.

        % Next step is to evaluate this function at ti_up, which is the current
        % time, to get the position is function would do.
        q_dir_adpt = adpt_fct(ti_up,ti+tx,T_up,qi_up,qf_up,vm,am,interpoly);
        % The difference of the adaption motion position and current position
        % of the final values of the linear part, is now used to shift the
        % adaption also in position level to the current values.
        delta_q = q_dir_adpt(1) - qf_1(1);
        delta_q_vec = zeros(3,1);
        delta_q_vec(1) = delta_q;

        % Next step is to calculate the real final values, which are the same
        % as the direct ones in velocity and acceleration level. But for
        % position level one needs to respect the delta_q shift.
        qf_real = qf_up - delta_q_vec;

        % To fit the interploator function at this final values again, a new
        % time shift is calculated 
        t_shift_up_inv = interpolator_1(qf_real(1), compute_traj_parameters(s0, v0, sf, v_inter_low, am));
        t_shift_up = t_shift_up_inv - (ti+tx+T_up) ;
        
        %%% Check if adaption is possible; Therefore the inverse functions
        % must be available.
        % If they return zero an adaption is not possible since start phase
        % is active; 
        % Another reason for no adaption is that the current acceleration 
        % is not zero.
        if t_inv == 0 || t_inv_up == 0|| t_shift_up_inv == 0 || qi(3)>0
            if start_opt == 1 % For delaying the start, the restart is used and set to the current value, if not done already
                adpt = false; 
                ti = 0;
                phase = 0;
                t_shift = t_shift_1;
                if restart == -1
                   restart = vm1; 
                end
            elseif start_opt == 2 % For delay and wait on update, the restart is set and ...
                adpt = false;
                ti = 0;
                phase = 0;
                t_shift = t_shift_1;
                adpt_blanking = vm; % ... the adpt_blanking variable is set to the current new velocity.
                if restart == -1
                   restart = vm1; 
                end
            end
        elseif start_opt >0 && (qf(3)~=0 || qf_up(3)~=0) %%% blanking for deceleration phase 
            if restart>=0
                adpt_blanking_end = restart;
            else
                adpt_blanking_end = vm1;
            end
            adpt = false; 
            ti = 0;
            phase = 0;
            t_shift = t_shift_1;
            restart = -1;
            adpt_blanking = -1;
        else
            % Reset variables
            restart = -1;
            adpt_blanking = -1;
        end  

        if adpt_blanking == vm % Only for startopt==2: If adaption would be possible, the code now waites for an update of vm.
            adpt = false;
            ti = 0;
        end
        
    end
end
    
%% This If runs only for one timestep!!!
% Rethink?! Phase 1 => Phase 2
if phase == 1 && t>=ti_up %End of phase 1
    if qi(2)<vf && vm<=0.5*(qf(2)+0.25*(3*vf+qi(2))) % If human stops or goes away meanwhile
        phase = 3;
        t_shift = t_shift_up;
    elseif qi(2)>vf && vm>=0.5*(qf(2)+0.25*(3*vf+qi(2)))  % If human stops or goes away meanwhile
        phase = 3;
        t_shift = t_shift_up;
    else
        phase = 2;
    end 
end

%% Here the actual motion is calculated
% Interpolates the values of pos,vel,acc (qv) with parameters and current time t 

if restart >=0
    [qdv, ipol_finished] = interpolator(t+t_shift, compute_traj_parameters(s0, v0, sf, restart, am));
elseif adpt_blanking_end >=0
    [qdv, ipol_finished] = interpolator(t+t_shift, compute_traj_parameters(s0, v0, sf, adpt_blanking_end, am));
else
    [qdv, ipol_finished] = interpolator(t+t_shift, compute_traj_parameters(s0, v0, sf, vm, am));
end  

%% If adaption motion needed
if adpt == true
    
    %%% Calc adaption motion
    ipol_finished=0;%Prevent finish command from old interpolator
    if phase == 1
        %%% opti_break
        T_est = T-(t-ti);
        if Tm<T_est
            opti_break_mem = 1; 
        end
        % accelerate till am
        qdv = adpt_fct(t,ti,T,qi,qf,vm,am,interpoly);
    elseif phase == 2
        %if time is equal than the finish time => adaption motion is complete
        %But it is aborted one timestep earlier, since the finish timestep
        %is already computed correctly by the standard interpolator.
        if t>=(ti+T-1*time_step)  
            adpt=false;     %If adaption finished => reset
            phase = 0;
            opti_break_mem = 0; 
            % Calculate finish time_step
            [qdv, ipol_finished] = interpolator(t+t_shift, compute_traj_parameters(s0, v0, sf, qf(2), am));
            if vm~=qf(2)  %If adaption is finished, but the vm value has changed again => restart from current velocity on
                restart = qf(2);
            else
                restart = -1;
            end            
        else
            %%% opti_break
            T_est = T-(t-ti);
            if Tm<T_est
                opti_break_mem = 1; 
            end
        
            % Adaption to vf velocity
            qdv = adpt_fct(t,ti,T,qi,qf,vm,am,interpoly); 
        end 
        
    elseif phase == 3
        % decelerate to 0 and reach v_inter_low
        
        tx = (T/4); %exact time shift 
        %if time is equal than the finish time => adaption motion is complete
        %But it is aborted one timestep earlier, since the finish timestep
        %is already computed correctly by the standard interpolator.
        if t>=(ti+tx+T_up-1*time_step) 
            adpt=false;     %If adaption finished => reset
            phase = 0;
            opti_break_mem = 0; 
            % Calculate finish time_step
            [qdv, ipol_finished] = interpolator(t+t_shift, compute_traj_parameters(s0, v0, sf, qf_up(2), am));
            restart = qf_up(2); %Imidiately Restart with the current velocity

        else
            %%% opti_break
            T_est = ((T/4)-(t-ti_up));
            if Tm<T_est
                opti_break_mem = 1; 
            end
        
            delta_q_vec = zeros(3,1);
            delta_q_vec(1) = delta_q; %Build delta_q vector
            % Evaluate adaption function, shift with tx in time and with shift delta_q in position level
            qdv = adpt_fct(t,ti+tx,T_up,qi_up,qf_up,vm,am,interpoly) - delta_q_vec;
        end
        
    end

end

%% Set output
if sf == s0          % No motion needed if start = end 
    qd = s0;         % => set initial values
    dqd = v0;
    ddqd = 0;  
else     
    qd = qdv(1);     % set output
    dqd = qdv(2);
    ddqd = qdv(3);        
end
opti_break = opti_break_mem;
vm1 = vm;  %remember current max velocity

end

function [qd,dqd,ddqd, ipol_finished] = calc_qd_f(t,s0,v0,sf,vm,am,T_scale,interpoly,time_step)
% This function calculates a one dimensional movement with a trapezodial 
% signal for velocity over time. Additionally it is able to adapt to shifts
% in the maximum allowed velocity.
%
% Inputs:
% t         current runtime
% s0        start value for motion in position
% v0        start value for motion in velocity
% sf        final value for motion in position
% vm        maximum allowed velocity
% am        maximum allowed acceleration
% T_scale   Scaling factor for duration of adaption
% interpoly Which interpolation to use
%
% Outputs:
% qd        disered position at current time
% dqd       disered velocity at current time
% ddqd      disered acceleration at current time
% ipol_finished 
%           motion is finished

%% Initialize persistent variables for adaption motion
persistent vm1 adpt ti qi qf T t_shift
if isempty(vm1)
    vm1 = vm;       %remembers the max velocity from last run
end
if isempty(adpt)
    adpt = false;   %stores if an adaption motion is activated
end
if isempty(ti)
    ti = 0;         %Initial time step for adaption motion
end
if isempty(qi)
    qi = zeros(3,1);%Initial values (pos,vel,acc) for adaption motion
end
if isempty(qf)
    qf = zeros(3,1);%Final values (pos,vel,acc) for adaption motion
end
if isempty(T)
    T = 0;          %Duration of adaption motion; tf = ti+T
end
if isempty(t_shift)
    t_shift = 0;    %Time distance with which the current reference motion is shifted
end


%% This If runs only for one timestep!!!
% If current max velocity is unequal to old one 
% Not directly at the beginning
% Dont start new while a adaption is still running, to prevent reset of
%   initial values
if abs(vm-vm1)>1e-3 && t>time_step && adpt==false                       
    adpt = true;          % Activate adaption
    ti = t;               % Set initial timestep to current step

    %%% inital set of position, velo, acceleration for adaption motion 
    % is the same as the old mogen would do (t_shift is not updated at
    % this time!)
    [qi, ~] = interpolator(ti+t_shift, compute_traj_parameters(s0, v0, sf, vm1, am));

    %%% computes the time shift for shifting the new motion to the end
    % point of the old motion. So at which time the new motion has
    % the same qd? Then calculate the time distance to the inital
    % time of the change in velocities
    % t_shift < 0 if new motion is faster (vm>vm1)
    % t_shift > 0 if new motion is slower (vm<vm1)
    % interpolator_1 is the inverse function of interpolator!
    t_shift = interpolator_1(qi(1), compute_traj_parameters(s0, v0, sf, vm, am)) - ti ;

    %%% Additional shift for adaption motion = Duration of adaption motion
    % Calculate duration of adaption
    if interpoly==0 
        T = 0;
        adpt = false;
    else
        T = T_calc(vm1,vm,am,T_scale,interpoly); 
    end

    %%% The additional shift for adaption motion is dependent on the
    % difference in the velocities. See report for details.
    t_shift  = t_shift+(T/2)*((vm1/vm)-1);

    %%% Calculate final values for adaption motion. Which are reached
    % at inital time plus duration of adaption and new time shift
    [qf, ~] = interpolator(ti+t_shift+T, compute_traj_parameters(s0, v0, sf, vm, am));

end

%% Here the actual motion is calculated
% Interpolates the values of pos,vel,acc (qv) with parameters and current time t    
[qdv, ipol_finished] = interpolator(t+t_shift, compute_traj_parameters(s0, v0, sf, vm, am));  

%% If adaption motion needed
if adpt == true 

    %%% calculate the adaption moition, which takes time from ti to
    % ti+T. t is the current runtime, _i initial values, _f final
    % values, _m maximum values

    qdv = adpt_fct(t,ti,T,qi,qf,vm,am,interpoly);

    % If time is equal than the finish time => adaption motion is complete
    % But it is aborted one timestep earlier, since the finish timestep
    % is already computed correctly by the standard interpolator.
    if t >= (ti+T-time_step)
        adpt = false;     % If adaption finished => reset
    end
end

%% Set output
if sf == s0          % No motion needed if start = end 
    qd = s0;         % => set initial values
    dqd = v0;
    ddqd = 0;  
else     
    qd = qdv(1);     % set output
    dqd = qdv(2);
    ddqd = qdv(3);        
end

vm1 = vm;  %remember current max velocity

end

function [T] = T_calc(v_current,v_goal,am,T_scale,interpoly)

    %%% Additional shift for adaption motion = Duration of adaption motion
    T_standard = abs(v_current-v_goal)/am;
    switch interpoly
        case 1
            T = T_standard*2.2;     %tanhlog
        case 2
            T = T_standard*(pi/2);  %Cosine version
        case 3
            T = T_standard;         %poly3
        case 4
            T = T_standard*1.5;     %poly4
        case 5
            T = T_standard*1.5;     %poly5
        case 7
            T = T_standard*1.75;    %poly7 
        otherwise
            T = T_standard;         %rest
    end

    % Scale Duration if needed
    T = T*T_scale;

end

function [T] = T_calc_a_scale(vc,vd,vm,v_eps,am,time_step,T_scale,interpoly)

a_min = (((vm*v_eps)/(am*time_step))-v_eps)/(vm-v_eps);
a_min = 1;%0.3;
T_standard = (abs(vc-vd))/(am*(a_min+(1-a_min)*((abs(vc-vd))/vm)));
    %%% Additional shift for adaption motion = Duration of adaption motion
    %T_standard = abs(v_current-v_goal)/am;
    switch interpoly
        case 1
            T = T_standard*2.2;    %tanhlog
        case 2
            T = T_standard*(pi/2);  %Cosine version
        case 3
            T = T_standard;        %poly3
        case 4
            T = T_standard*1.5; %poly4
        case 5
            T = T_standard*1.5;        %poly5 1,5
        case 7
            T = T_standard*1.75;        %poly7 
        otherwise
            T = T_standard;        %rest
    end

    % Scale Duration if needed
     T = T*T_scale;

end

function [qdv] = adpt_fct(t,ti,T,qi,qf,vm,am,interpoly)
    
    %%% calculate the adaption moition, which takes time from ti to
    % ti+T. t is the current runtime, _i initial values, _f final
    % values, _m maximum values

    switch interpoly 
        case 0
            qdv = qf;   %No adaption
        case 1
            qdv = tanhlog(t,ti,T,qi,qf,vm,am);      %tanhlog
        case 2
            qdv = cosine(t,ti,T,qi,qf,vm,am);       %Cosine version
        case 3
            qdv = poly3(t,ti,T,qi,qf,vm,am);        %poly3
        case 4
            qdv = poly4(t,ti,T,qi,qf,vm,am);        %poly4
        case 5
            qdv = poly5_end(t,ti,T,qi,qf,vm,am);        %poly5; Dont use poly5 function: Has a bug?!
        case 6
            qdv = poly6(t,ti,T,qi,qf,vm,am);        %poly6 
        case 7
            qdv = poly7(t,ti,T,qi,qf,vm,am);        %poly7 
        case 8
            qdv = poly4_mean(t,ti,T,qi,qf,vm,am);   %poly4_mean 
        case 9
            qdv = poly5_2mean(t,ti,T,qi,qf,vm,am);  %poly5_2mean 
        case 10
            qdv = tanhmean(t,ti,T,qi,qf,vm,am);     %tanhmean 
        otherwise
            error('Unknown adaption motion');       %rest
    end
    
end

function [T2,T3,ti3,qi3,qf3,delta_q3,t_shift3,error_state] = calc_g_update_fct(vd_up,v_delta_stop,qi1,ti2,parameter2,am,T_scale,interpoly,s0, v0, sf,start_opt,vm,v_eps,time_step)
%%% In this function the trajectory is calculated, with all parameters especially
%%% for phase 3.
% While calc an errors could occur due to acceleration or deceleration
% phase, this is reflected in error_state as following:
% 0 = No errors
% 1 = Error due to too early start = acceleration phase
% 2 = Error due to collision with deceleration phase

%init all 0 because of return of error_state if adaption not possible.
T2=0;
T3=0;
ti3=0;
qi3=zeros(3,1);
qf3=zeros(3,1);
delta_q3=0;
t_shift3=0;
error_state=0;

% calc final velocity of phase 2
v_final2 = vd_up+v_delta_stop; %target minus stopping
T2 = ((v_final2-parameter2(2))/parameter2(3));% Exact Duration of phase 2

% calculate what linear part would do at its end = final value of phase 2
qf2 = zeros(3,1); %final value of phase 2
qf2(1) = 0.5*parameter2(3)*T2^2+parameter2(2)*T2+parameter2(1);
qf2(2) = parameter2(3)*T2+parameter2(2);
qf2(3) = parameter2(3);

% Parameters for Phase 3 = stopping adaption part
ti3 = ti2 + T2; % initial time for phase 3

% set virtual starting point of phase 3; position wrong, but velocity correct
qi3 = [qi1(1);vd_up+2*v_delta_stop;0]; 

% This not directly the duration of phase 3, because of the virtual part
T3 = T_calc(qi3(2),vd_up,am,T_scale,interpoly); 
%T3 = T_calc_a_scale(qi3(2),vd_up,vm,v_eps,am,time_step,T_scale,interpoly); 
tx = -T3/2; %exact time shift tx,  between ti3 and virtual start point of adaption in phase 3

% Calculate a time shift for the interpolator, from qi3 on, with
% current vm as goal
t_shift_inter_inv = interpolator_1(qi3(1), compute_traj_parameters(s0, v0, sf, vd_up, am));
% check if inverse interpolator was evaluatable
if start_opt>0 && t_shift_inter_inv==0
    error_state = 1;
    return
elseif start_opt>0 && t_shift_inter_inv==-1
    error_state = 2;
    return
end
t_shift_inter = t_shift_inter_inv - (ti3+tx);
t_shift_inter = t_shift_inter+(T3/2)*((qi3(2)/vd_up)-1);

% Also calculate final values of phase 3
[qf3, ~] = interpolator(ti3+tx+t_shift_inter+T3, compute_traj_parameters(s0, v0, sf, vd_up, am));
% check if interpolator is in acc/dec phase
if start_opt>0 && qf3(3)>0
    error_state = 1;
    return
elseif start_opt>0 && qf3(3)<0
    error_state = 2;
    return
end

% From now on this initial and final values are used in the adaption
% function for the phase 3. This function is also shifted in time
% with the tx value, so starting time is ti3+tx.

% Next step is to evaluate this function at ti3, which is the end of
% the linear part. 
q_inter = adpt_fct(ti3,ti3+tx,T3,qi3,qf3,vd_up,am,interpoly);

% The difference of the adaption motion position and position
% of the final values of the linear part, is now used to shift the
% adaption also in position level to the correct values.
delta_q3 = q_inter(1) - qf2(1);
delta_q_vec = zeros(3,1);
delta_q_vec(1) = delta_q3;

% Next step is to calculate the real final values, which are the same
% as the direct ones in velocity and acceleration level. But for
% position level one needs to respect the delta_q shift.
qf_real = qf3 - delta_q_vec;

% To fit the interpolator function at this final values again, a new
% time shift is calculated, which is activated from phase 3 on
t_shift3_inv = interpolator_1(qf_real(1), compute_traj_parameters(s0, v0, sf, vd_up, am));
% check if inverse interpolator was evaluatable
if start_opt>0 && t_shift3_inv==0
    error_state = 1;
    return
elseif start_opt>0 && t_shift3_inv==-1
    error_state = 2;
    return
end
t_shift3 = t_shift3_inv - (ti3+tx+T3) ;
    
end

function [qv] = poly3(t,ti,T,qvi,qvf,dqm,ddqm)
%POLY3 computes a polynomial trajectory of degree 3 between initial (_i) 
%values and final (_f) values of position q, velocity dq and accelerataion
%ddq. Taken from Melchiorri presentation page 19

qi = qvi(1);      %split input vectors in pos,vel,acc
dqi = qvi(2);
ddqi = qvi(3);
qf = qvf(1);
dqf = qvf(2);
ddqf = qvf(3);
      
% current duration of motion dt
dt = t-ti;                      

% compute coefficients
a0 = qi;
a1 = dqi;
a2 = (-3*(qi-qf)-(2*dqi+dqf)*T)/(T^2);
a3 = (2*(qi-qf)+(dqi+dqf)*T)/(T^3);

% compute pos,vel,acc desired (_d)
qd = a0+a1*dt+a2*dt^2+a3*dt^3;
dqd = a1+2*a2*dt+3*a3*dt^2;
ddqd = 2*a2+6*a3*dt;

qv = [qd;dqd;ddqd]; %Send values back

end

function [qv] = poly4(t,ti,T,qvi,qvf,dqm,ddqm)
%POLY4 computes a polynomial trajectory of degree 4 between initial (_i) 
%values and final (_f) values of position q, velocity dq and accelerataion
%ddq. inspired by old function in here

qi = qvi(1);      %split input vectors in pos,vel,acc
dqi = qvi(2);
ddqi = qvi(3);
qf = qvf(1);
dqf = qvf(2);
ddqf = qvf(3);
      
% current duration of motion dt
dt = t-ti;                      

% a2 = 0;
% a3 = -4/9*ddqm^2/(dqi-dqm);
% a4 = -4/27*ddqm^3/(dqi-dqm)^2;
a2 = 0;
a3 = -4/9*ddqm^2/abs(dqi-dqf);
a4 = 4/27*ddqm^3/abs(dqi-dqf)^2;

a0 = qi;
a1 = dqi;
% a2 = 0.5*ddqi;
% a3 = (4*(qf-qi)-(dqf+3*dqi)*T-ddqi*(T^2))/(T^3);
% a4 = (3*(qi-qf)+(dqf+2*dqi)*T+0.5*ddqi*(T^2))/(T^4);

% compute pos,vel,acc desired (_d)
qd = (a4*dt^4+a3*dt^3+a2*dt^2+a1*dt+a0);
dqd = 4*a4*dt^3+3*a3*dt^2+2*a2*dt+a1;
ddqd = 12*a4*dt^2+6*a3*dt+2*a2;

qv = [qd;dqd;ddqd]; %Send values back

end

function [qv] = poly4_mean(t,ti,T,qvi,qvf,dqm,ddqm)
%POLY4 computes a polynomial trajectory of degree 4 between initial (_i) 
%values and final (_f) values of position q, velocity dq and accelerataion
%ddq with mean velocity at T/2. self made

qi = qvi(1);      %split input vectors in pos,vel,acc
dqi = qvi(2);
ddqi = qvi(3);
qf = qvf(1);
dqf = qvf(2);
ddqf = qvf(3);
      
% current duration of motion dt
dt = t-ti;                     

b = [qi dqi qf dqf 0.5*(dqi+dqf)]';

M_inv = [...
       1,     0,      0,          0,           0;
       0,     1,      0,          0,           0;
   6/T^2,  -2/T, -6/T^2,    5/(4*T),    27/(4*T);
 -16/T^3, 1/T^2, 16/T^3, -7/(2*T^2), -27/(2*T^2);
   9/T^4,     0, -9/T^4,  9/(4*T^3),  27/(4*T^3)];

a = M_inv * b;

% compute pos,vel,acc desired (_d)

qd = a(1)+a(2)*dt+a(3)*dt^2+a(4)*dt^3+a(5)*dt^4;
dqd = a(2)+2*a(3)*dt+3*a(4)*dt^2+4*a(5)*dt^3;
ddqd = 2*a(3)+6*a(4)*dt+12*a(5)*dt^2;

qv = [qd;dqd;ddqd]; %Send values back

end

function [qv] = poly5(t,ti,T,qvi,qvf,dqm,ddqm)
%POLY5 computes a polynomial trajectory of degree 5 between initial (_i) 
%values and final (_f) values of position q, velocity dq and accelerataion
%ddq. Taken from Melchiorri presentation page 25

qi = qvi(1);      %split input vectors in pos,vel,acc
dqi = qvi(2);
ddqi = qvi(3);
qf = qvf(1);
dqf = qvf(2);
ddqf = qvf(3);
      
% current duration of motion dt
dt = t-ti;                      

% compute coefficients
a0 = qi;
a1 = dqi;
a2 = 0.5*ddqi;
a3 = (20*(qf-qi)-(8*dqf+12*dqi)*T-(3*ddqf-ddqi)*T^2)/(2*T^3);
a4 = (30*(qi-qf)+(14*dqf+16*dqi)*T+(3*ddqf-2*ddqi)*T^2)/(2*T^4);
a5 = (12*(qf-qi)-6*(dqf+dqi)*T-(ddqf-ddqi)*T^2)/(2*T^5);
% compute pos,vel,acc desired (_d)
qd = a0+a1*dt+a2*dt^2+a3*dt^3+a4*dt^4+a5*dt^5;
dqd = a1+2*a2*dt+3*a3*dt^2+4*a4*dt^3+5*a5*dt^4;
ddqd = 2*a2+6*a3*dt+12*a4*dt^2+20*a5*dt^3;

qv = [qd;dqd;ddqd]; %Send values back

end

function [qv] = poly5_end(t,ti,T,qvi,qvf,dqm,ddqm)
%POLY5 self made, other poly5 has a bug somehow

qi = qvi(1);      %split input vectors in pos,vel,acc
dqi = qvi(2);
ddqi = qvi(3);
qf = qvf(1);
dqf = qvf(2);
ddqf = qvf(3);
      
% current duration of motion dt
dt = t-ti;                      
 
a = [...
                                                                                  qi
                                                                                 dqi
                                                                              ddqi/2
 ddqf/(2*T) - (3*ddqi)/(2*T) - (4*dqf)/T^2 - (6*dqi)/T^2 + (10*qf)/T^3 - (10*qi)/T^3
 (3*ddqi)/(2*T^2) - ddqf/T^2 + (7*dqf)/T^3 + (8*dqi)/T^3 - (15*qf)/T^4 + (15*qi)/T^4
   ddqf/(2*T^3) - ddqi/(2*T^3) - (3*dqf)/T^4 - (3*dqi)/T^4 + (6*qf)/T^5 - (6*qi)/T^5];
 


% compute pos,vel,acc desired (_d)

qd = a(1)+a(2)*dt+a(3)*dt^2+a(4)*dt^3+a(5)*dt^4+a(6)*dt^5;
dqd = a(2)+2*a(3)*dt+3*a(4)*dt^2+4*a(5)*dt^3+5*a(6)*dt^4;
ddqd = 2*a(3)+6*a(4)*dt+12*a(5)*dt^2+20*a(6)*dt^3;

qv = [qd;dqd;ddqd]; %Send values back

end

function [qv] = poly5_2mean(t,ti,T,qvi,qvf,dqm,ddqm)
%POLY5 computes a polynomial trajectory of degree 5 between initial (_i) 
%values and final (_f) values of position q, velocity dq and accelerataion
%ddq with 2*mean steps at T/3 and 2T/3. self made

qi = qvi(1);      %split input vectors in pos,vel,acc
dqi = qvi(2);
ddqi = qvi(3);
qf = qvf(1);
dqf = qvf(2);
ddqf = qvf(3);
      
% current duration of motion dt
dt = t-ti;                      

% compute coefficients
b = [qi dqi qf dqf 0.5*(dqi+dqf)+(1/6)*(dqi-dqf) 0.5*(dqi+dqf)+(1/6)*(dqi-dqf)]';

M_inv = [...
        1,          0,        0,           0,            0,           0;
        0,          1,        0,           0,            0,           0;
  -30/T^2,  -13/(2*T),   30/T^2,   -13/(4*T),    -27/(4*T),   -27/(2*T);
  110/T^3, 67/(4*T^2), -110/T^3,  49/(4*T^2),  135/(4*T^2), 189/(4*T^2);
 -135/T^4,    -18/T^3,  135/T^4, -63/(4*T^3), -189/(4*T^3),     -54/T^3;
   54/T^5, 27/(4*T^4),  -54/T^5,  27/(4*T^4),   81/(4*T^4),  81/(4*T^4)];

a = M_inv * b;

% compute pos,vel,acc desired (_d)

qd = a(1)+a(2)*dt+a(3)*dt^2+a(4)*dt^3+a(5)*dt^4+a(6)*dt^5;
dqd = a(2)+2*a(3)*dt+3*a(4)*dt^2+4*a(5)*dt^3+5*a(6)*dt^4;
ddqd = 2*a(3)+6*a(4)*dt+12*a(5)*dt^2+20*a(6)*dt^3;

qv = [qd;dqd;ddqd]; %Send values back

end

function [qv] = poly6(t,ti,T,qvi,qvf,dqm,ddqm)
%POLY6 computes a polynomial trajectory of degree 6 between initial (_i) 
%values and final (_f) values of position q, velocity dq and accelerataion
%ddq with mean velocity at T/3. self made

qi = qvi(1);      %split input vectors in pos,vel,acc
dqi = qvi(2);
ddqi = qvi(3);
qf = qvf(1);
dqf = qvf(2);
ddqf = qvf(3);

% current duration of motion dt
dt = t-ti;                      

% compute coefficients
b = [qi dqi 0.5*ddqi qf dqf ddqf 0.5*(dqi+dqf)]';

M_inv = [...
       1,      0,      0,       0,           0,          0,            0;
       0,      1,      0,       0,           0,          0,            0;
       0,      0,      1,       0,           0,          0,            0;
  20/T^3, -6/T^2,   -4/T, -20/T^3,  23/(4*T^2),   -1/(2*T),   81/(4*T^2);
 -75/T^4,  8/T^3,  6/T^2,  75/T^4, -89/(4*T^3),      2/T^2, -243/(4*T^3);
  84/T^5, -3/T^4, -4/T^3, -84/T^5, 105/(4*T^4), -5/(2*T^3),  243/(4*T^4);
 -30/T^6,      0,  1/T^4,  30/T^6, -39/(4*T^5),      1/T^4,  -81/(4*T^5)];

a = M_inv * b;

% compute pos,vel,acc desired (_d)

qd = a(1)+a(2)*dt+a(3)*dt^2+a(4)*dt^3+a(5)*dt^4+a(6)*dt^5+a(7)*dt^6;
dqd = a(2)+2*a(3)*dt+3*a(4)*dt^2+4*a(5)*dt^3+5*a(6)*dt^4+6*a(7)*dt^5;
ddqd = 2*a(3)+6*a(4)*dt+12*a(5)*dt^2+20*a(6)*dt^3+30*a(7)*dt^4;

qv = [qd;dqd;ddqd]; %Send values back

end

function [qv] = poly7(t,ti,T,qvi,qvf,dqm,ddqm)
%POLY7 computes a polynomial trajectory of degree 7 between initial (_i) 
%values and final (_f) values of position q, velocity dq, accelerataion
%ddq and jerk dddq. self made

qi = qvi(1);      %split input vectors in pos,vel,acc
dqi = qvi(2);
ddqi = qvi(3);
dddqi = 0;
qf = qvf(1);
dqf = qvf(2);
ddqf = qvf(3);
dddqf = 0;

% current duration of motion dt
dt = t-ti;                      

% compute coefficients
 
a = [...
                                                                                                                                                                            conj(qi)
                                                                                                                                                                           conj(dqi)
                                                                                                                                                                        conj(ddqi)/2
                                                                                                                                                                       conj(dddqi)/6
           (5*conj(ddqf))/(2*T^2) - (2*conj(dddqi))/(3*T) - conj(dddqf)/(6*T) - (5*conj(ddqi))/T^2 - (15*conj(dqf))/T^3 - (20*conj(dqi))/T^3 + (35*conj(qf))/T^4 - (35*conj(qi))/T^4
                  conj(dddqf)/(2*T^2) + conj(dddqi)/T^2 - (7*conj(ddqf))/T^3 + (10*conj(ddqi))/T^3 + (39*conj(dqf))/T^4 + (45*conj(dqi))/T^4 - (84*conj(qf))/T^5 + (84*conj(qi))/T^5
 (13*conj(ddqf))/(2*T^4) - (2*conj(dddqi))/(3*T^3) - conj(dddqf)/(2*T^3) - (15*conj(ddqi))/(2*T^4) - (34*conj(dqf))/T^5 - (36*conj(dqi))/T^5 + (70*conj(qf))/T^6 - (70*conj(qi))/T^6
               conj(dddqf)/(6*T^4) + conj(dddqi)/(6*T^4) - (2*conj(ddqf))/T^5 + (2*conj(ddqi))/T^5 + (10*conj(dqf))/T^6 + (10*conj(dqi))/T^6 - (20*conj(qf))/T^7 + (20*conj(qi))/T^7];
 


% compute pos,vel,acc desired (_d)

qd = a(1)+a(2)*dt+a(3)*dt^2+a(4)*dt^3+a(5)*dt^4+a(6)*dt^5+a(7)*dt^6+a(8)*dt^7;
dqd = a(2)+2*a(3)*dt+3*a(4)*dt^2+4*a(5)*dt^3+5*a(6)*dt^4+6*a(7)*dt^5+7*a(8)*dt^6;
ddqd = 2*a(3)+6*a(4)*dt+12*a(5)*dt^2+20*a(6)*dt^3+30*a(7)*dt^4+42*a(8)*dt^5;

qv = [qd;dqd;ddqd]; %Send values back

end

function [qv] = cosine(t,ti,T,qvi,qvf,dqm,ddqm)
%COSINE computes a cosine trajectory between initial (_i) 
%values and final (_f) values of position q, velocity dq and accelerataion
%ddq with respect to the maximum values (_m). t is the current runtime

qi = qvi(1);      %split input vectors in pos,vel,acc
dqi = qvi(2);
ddqi = qvi(3);
qf = qvf(1);
dqf = qvf(2);
ddqf = qvf(3);
      
% often needed values

%T = (pi*abs(dqf-dqi))/(2*ddqm); % total duration of motion T (with am)
%T = abs((2*(qf-qi))/(dqi-dqf));
dt = t-ti;                      % current duration of motion dt

%cm = (T/(2*pi))*(dqm-(1/T)*(qf-qi));
c = qi-0.5*(dqi+dqf)*ti;
%cn = qf-0.5*(dqi+dqf)*(ti+T);
%c = cn + 0.5*(1+cos((pi/T)*dt))*(ca-cn);


% if t<(ti+(T/2))
%     c = qi - 0.5*(dqi+dqf)*ti;
% else
%     c = qf - 0.5*(((dqi+dqf)/2)+dqf)*tf;
% end

%c = (qi+qf)/2 - 0.5*(dqi+dqf)*(ti+(T/2)) - 0.5*(dqi-dqf)*(T/pi);
% compute pos,vel,acc desired (_d)
%qd = qi + (1/T)*(qf-qi)*dt + cm*sin(((2*pi)/T)*dt);
qd = 0.5*(dqi+dqf)*t + 0.5*(T/pi)*(dqi-dqf)*sin((pi/T)*dt) + c;
dqd = 0.5*(dqi+dqf) + 0.5*(dqi-dqf)*cos((pi/T)*dt);
ddqd = -0.5*(pi/T)*(dqi-dqf)*sin((pi/T)*dt);

qv = [qd;dqd;ddqd]; %Send values back

end

function [qv] = tanhmean(t,ti,T,qvi,qvf,dqm,ddqm)
%TANHMEAN computes a tanh trajectory between initial (_i) 
%values and final (_f) values of position q, velocity dq and accelerataion
%ddq with respect to the maximum values (_m). t is the current runtime
%selfmade

qi = qvi(1);      %split input vectors in pos,vel,acc
dqi = qvi(2);
ddqi = qvi(3);
qf = qvf(1);
dqf = qvf(2);
ddqf = qvf(3);
      
% current duration of motion dt
dt = t-ti;                      
t_norm = dt/T;
theta = 4;

qd = 0.5*(1/theta)*(dqf-dqi)*log(cosh(theta*(t_norm-0.5))) ...
     + 0.5*(dqi+dqf)*t_norm ...
     + qf - 0.5*(1/theta)*(dqf-dqi)*log(cosh(0.5*theta));
     %+ qi - 0.5*(1/theta)*(dqf-dqi)*log(cosh(-0.5*theta));
dqd = 0.5*(dqi+dqf) + 0.5*(dqf-dqi)*tanh(theta*(t_norm-0.5));
ddqd = 0.5*theta*(dqf-dqi)*sech(t_norm-0.5)^2;

qv = [qd;dqd;ddqd]; %Send values back

end

function [qv] = tanhlog(t,ti,T,qvi,qvf,dqm,ddqm)
%TANHLOG computes a tanh-log trajectory between initial (_i) 
%values and final (_f) values of position q, velocity dq and accelerataion
%ddq with respect to the maximum values (_m). t is the current runtime
%taken from Internet

% Threshold for checks
th = 1e-6;

% current duration of motion dt
dt = t-ti;  

% tanhlog cannot compute first and last value, due to ln(0) problems.
% So if tanhlog is evaluated around zero and below, qvi is returned.
% And if tanhlog is evaluated at a time near or higher than the planned
% duration qvf is returned.
if dt<th
    qv = qvi;
elseif T-dt<th
    qv = qvf;
else
    qi = qvi(1);      %split input vectors in pos,vel,acc
    dqi = qvi(2);
    ddqi = qvi(3);
    qf = qvf(1);
    dqf = qvf(2);
    ddqf = qvf(3);
   
    a = dqi;
    b = qi;      
    c = dqf;
    d = qf-dqf*T;
    k = d-b;
    
    if abs(k)>th
        x = (a*dt+b-c*dt-d+k)/(2*k);
        if x>th && x<(1-th)
            w = (tanh(((log(1-x))^2-(log(x))^2)/3)+1)/2;
            p = tanh((log(2-x)-log(x))*(1-(1/sqrt(2))*(log(2-x)+log(x))))+2*x-1;
            q = tanh((log(x+1)-log(1-x))*(1-(1/sqrt(2))*(log(1-x)+log(x+1))));
            s = p*(1-w)+q*w;

            qd = k*s+c*dt+d-k;

            dqd = dqf + (qi - qf + T*dqf)*((tanh(log((dqf*dt - dqi*dt)/(2*qi - 2*qf + 2*T*dqf))^2/3 - log(1 - (dqf*dt - dqi*dt)/(2*qi - 2*qf + 2*T*dqf))^2/3)/2 + 1/2)*((((2^(1/2)*(log(2 - (dqf*dt - dqi*dt)/(2*qi - 2*qf + 2*T*dqf)) + log((dqf*dt - dqi*dt)/(2*qi - 2*qf + 2*T*dqf))))/2 - 1)*((dqf - dqi)/(dqf*dt - dqi*dt) - (dqf - dqi)/(((dqf*dt - dqi*dt)/(2*qi - 2*qf + 2*T*dqf) - 2)*(2*qi - 2*qf + 2*T*dqf))) - (2^(1/2)*(log(2 - (dqf*dt - dqi*dt)/(2*qi - 2*qf + 2*T*dqf)) - log((dqf*dt - dqi*dt)/(2*qi - 2*qf + 2*T*dqf)))*((dqf - dqi)/(dqf*dt - dqi*dt) + (dqf - dqi)/(((dqf*dt - dqi*dt)/(2*qi - 2*qf + 2*T*dqf) - 2)*(2*qi - 2*qf + 2*T*dqf))))/2)*(tanh((log(2 - (dqf*dt - dqi*dt)/(2*qi - 2*qf + 2*T*dqf)) - log((dqf*dt - dqi*dt)/(2*qi - 2*qf + 2*T*dqf)))*((2^(1/2)*(log(2 - (dqf*dt - dqi*dt)/(2*qi - 2*qf + 2*T*dqf)) + log((dqf*dt - dqi*dt)/(2*qi - 2*qf + 2*T*dqf))))/2 - 1))^2 - 1) - (2*(dqf - dqi))/(2*qi - 2*qf + 2*T*dqf)) - (tanh(((2^(1/2)*(log((dqf*dt - dqi*dt)/(2*qi - 2*qf + 2*T*dqf) + 1) + log(1 - (dqf*dt - dqi*dt)/(2*qi - 2*qf + 2*T*dqf))))/2 - 1)*(log((dqf*dt - dqi*dt)/(2*qi - 2*qf + 2*T*dqf) + 1) - log(1 - (dqf*dt - dqi*dt)/(2*qi - 2*qf + 2*T*dqf))))^2 - 1)*(tanh(log((dqf*dt - dqi*dt)/(2*qi - 2*qf + 2*T*dqf))^2/3 - log(1 - (dqf*dt - dqi*dt)/(2*qi - 2*qf + 2*T*dqf))^2/3)/2 - 1/2)*(((2^(1/2)*(log((dqf*dt - dqi*dt)/(2*qi - 2*qf + 2*T*dqf) + 1) + log(1 - (dqf*dt - dqi*dt)/(2*qi - 2*qf + 2*T*dqf))))/2 - 1)*((dqf - dqi)/(((dqf*dt - dqi*dt)/(2*qi - 2*qf + 2*T*dqf) - 1)*(2*qi - 2*qf + 2*T*dqf)) - (dqf - dqi)/(((dqf*dt - dqi*dt)/(2*qi - 2*qf + 2*T*dqf) + 1)*(2*qi - 2*qf + 2*T*dqf))) - (2^(1/2)*(log((dqf*dt - dqi*dt)/(2*qi - 2*qf + 2*T*dqf) + 1) - log(1 - (dqf*dt - dqi*dt)/(2*qi - 2*qf + 2*T*dqf)))*((dqf - dqi)/(((dqf*dt - dqi*dt)/(2*qi - 2*qf + 2*T*dqf) - 1)*(2*qi - 2*qf + 2*T*dqf)) + (dqf - dqi)/(((dqf*dt - dqi*dt)/(2*qi - 2*qf + 2*T*dqf) + 1)*(2*qi - 2*qf + 2*T*dqf))))/2) + (tanh(((2^(1/2)*(log((dqf*dt - dqi*dt)/(2*qi - 2*qf + 2*T*dqf) + 1) + log(1 - (dqf*dt - dqi*dt)/(2*qi - 2*qf + 2*T*dqf))))/2 - 1)*(log((dqf*dt - dqi*dt)/(2*qi - 2*qf + 2*T*dqf) + 1) - log(1 - (dqf*dt - dqi*dt)/(2*qi - 2*qf + 2*T*dqf))))*((2*log((dqf*dt - dqi*dt)/(2*qi - 2*qf + 2*T*dqf))*(dqf - dqi))/(3*(dqf*dt - dqi*dt)) - (2*log(1 - (dqf*dt - dqi*dt)/(2*qi - 2*qf + 2*T*dqf))*(dqf - dqi))/(3*((dqf*dt - dqi*dt)/(2*qi - 2*qf + 2*T*dqf) - 1)*(2*qi - 2*qf + 2*T*dqf)))*(tanh(log((dqf*dt - dqi*dt)/(2*qi - 2*qf + 2*T*dqf))^2/3 - log(1 - (dqf*dt - dqi*dt)/(2*qi - 2*qf + 2*T*dqf))^2/3)^2 - 1))/2 - (((2*log((dqf*dt - dqi*dt)/(2*qi - 2*qf + 2*T*dqf))*(dqf - dqi))/(3*(dqf*dt - dqi*dt)) - (2*log(1 - (dqf*dt - dqi*dt)/(2*qi - 2*qf + 2*T*dqf))*(dqf - dqi))/(3*((dqf*dt - dqi*dt)/(2*qi - 2*qf + 2*T*dqf) - 1)*(2*qi - 2*qf + 2*T*dqf)))*(tanh(log((dqf*dt - dqi*dt)/(2*qi - 2*qf + 2*T*dqf))^2/3 - log(1 - (dqf*dt - dqi*dt)/(2*qi - 2*qf + 2*T*dqf))^2/3)^2 - 1)*(tanh((log(2 - (dqf*dt - dqi*dt)/(2*qi - 2*qf + 2*T*dqf)) - log((dqf*dt - dqi*dt)/(2*qi - 2*qf + 2*T*dqf)))*((2^(1/2)*(log(2 - (dqf*dt - dqi*dt)/(2*qi - 2*qf + 2*T*dqf)) + log((dqf*dt - dqi*dt)/(2*qi - 2*qf + 2*T*dqf))))/2 - 1)) - (2*(dqf*dt - dqi*dt))/(2*qi - 2*qf + 2*T*dqf) + 1))/2);

            ddqd = -(qi - qf + T*dqf)*(((tanh(log((dqf*dt - dqi*dt)/(2*qi - 2*qf + 2*T*dqf))^2/3 - log(1 - (dqf*dt - dqi*dt)/(2*qi - 2*qf + 2*T*dqf))^2/3)^2 - 1)*(tanh((log(2 - (dqf*dt - dqi*dt)/(2*qi - 2*qf + 2*T*dqf)) - log((dqf*dt - dqi*dt)/(2*qi - 2*qf + 2*T*dqf)))*((2^(1/2)*(log(2 - (dqf*dt - dqi*dt)/(2*qi - 2*qf + 2*T*dqf)) + log((dqf*dt - dqi*dt)/(2*qi - 2*qf + 2*T*dqf))))/2 - 1)) - (2*(dqf*dt - dqi*dt))/(2*qi - 2*qf + 2*T*dqf) + 1)*((2*(dqf - dqi)^2)/(3*(dqf*dt - dqi*dt)^2) - (2*(dqf - dqi)^2)/(3*((dqf*dt - dqi*dt)/(2*qi - 2*qf + 2*T*dqf) - 1)^2*(2*qi - 2*qf + 2*T*dqf)^2) - (2*log((dqf*dt - dqi*dt)/(2*qi - 2*qf + 2*T*dqf))*(dqf - dqi)^2)/(3*(dqf*dt - dqi*dt)^2) + (2*log(1 - (dqf*dt - dqi*dt)/(2*qi - 2*qf + 2*T*dqf))*(dqf - dqi)^2)/(3*((dqf*dt - dqi*dt)/(2*qi - 2*qf + 2*T*dqf) - 1)^2*(2*qi - 2*qf + 2*T*dqf)^2)))/2 - (tanh(((2^(1/2)*(log((dqf*dt - dqi*dt)/(2*qi - 2*qf + 2*T*dqf) + 1) + log(1 - (dqf*dt - dqi*dt)/(2*qi - 2*qf + 2*T*dqf))))/2 - 1)*(log((dqf*dt - dqi*dt)/(2*qi - 2*qf + 2*T*dqf) + 1) - log(1 - (dqf*dt - dqi*dt)/(2*qi - 2*qf + 2*T*dqf))))*(tanh(log((dqf*dt - dqi*dt)/(2*qi - 2*qf + 2*T*dqf))^2/3 - log(1 - (dqf*dt - dqi*dt)/(2*qi - 2*qf + 2*T*dqf))^2/3)^2 - 1)*((2*(dqf - dqi)^2)/(3*(dqf*dt - dqi*dt)^2) - (2*(dqf - dqi)^2)/(3*((dqf*dt - dqi*dt)/(2*qi - 2*qf + 2*T*dqf) - 1)^2*(2*qi - 2*qf + 2*T*dqf)^2) - (2*log((dqf*dt - dqi*dt)/(2*qi - 2*qf + 2*T*dqf))*(dqf - dqi)^2)/(3*(dqf*dt - dqi*dt)^2) + (2*log(1 - (dqf*dt - dqi*dt)/(2*qi - 2*qf + 2*T*dqf))*(dqf - dqi)^2)/(3*((dqf*dt - dqi*dt)/(2*qi - 2*qf + 2*T*dqf) - 1)^2*(2*qi - 2*qf + 2*T*dqf)^2)))/2 - (tanh(log((dqf*dt - dqi*dt)/(2*qi - 2*qf + 2*T*dqf))^2/3 - log(1 - (dqf*dt - dqi*dt)/(2*qi - 2*qf + 2*T*dqf))^2/3)/2 + 1/2)*((tanh((log(2 - (dqf*dt - dqi*dt)/(2*qi - 2*qf + 2*T*dqf)) - log((dqf*dt - dqi ...
                *dt)/(2*qi - 2*qf + 2*T*dqf)))*((2^(1/2)*(log(2 - (dqf*dt - dqi*dt)/(2*qi - 2*qf + 2*T*dqf)) + log((dqf*dt - dqi*dt)/(2*qi - 2*qf + 2*T*dqf))))/2 - 1))^2 - 1)*((2^(1/2)*(log(2 - (dqf*dt - dqi*dt)/(2*qi - 2*qf + 2*T*dqf)) - log((dqf*dt - dqi*dt)/(2*qi - 2*qf + 2*T*dqf)))*((dqf - dqi)^2/(dqf*dt - dqi*dt)^2 + (dqf - dqi)^2/(((dqf*dt - dqi*dt)/(2*qi - 2*qf + 2*T*dqf) - 2)^2*(2*qi - 2*qf + 2*T*dqf)^2)))/2 - ((dqf - dqi)^2/(dqf*dt - dqi*dt)^2 - (dqf - dqi)^2/(((dqf*dt - dqi*dt)/(2*qi - 2*qf + 2*T*dqf) - 2)^2*(2*qi - 2*qf + 2*T*dqf)^2))*((2^(1/2)*(log(2 - (dqf*dt - dqi*dt)/(2*qi - 2*qf + 2*T*dqf)) + log((dqf*dt - dqi*dt)/(2*qi - 2*qf + 2*T*dqf))))/2 - 1) + 2^(1/2)*((dqf - dqi)/(dqf*dt - dqi*dt) + (dqf - dqi)/(((dqf*dt - dqi*dt)/(2*qi - 2*qf + 2*T*dqf) - 2)*(2*qi - 2*qf + 2*T*dqf)))*((dqf - dqi)/(dqf*dt - dqi*dt) - (dqf - dqi)/(((dqf*dt - dqi*dt)/(2*qi - 2*qf + 2*T*dqf) - 2)*(2*qi - 2*qf + 2*T*dqf)))) + 2*tanh((log(2 - (dqf*dt - dqi*dt)/(2*qi - 2*qf + 2*T*dqf)) - log((dqf*dt - dqi*dt)/(2*qi - 2*qf + 2*T*dqf)))*((2^(1/2)*(log(2 - (dqf*dt - dqi*dt)/(2*qi - 2*qf + 2*T*dqf)) + log((dqf*dt - dqi*dt)/(2*qi - 2*qf + 2*T*dqf))))/2 - 1))*(((2^(1/2)*(log(2 - (dqf*dt - dqi*dt)/(2*qi - 2*qf + 2*T*dqf)) + log((dqf*dt - dqi*dt)/(2*qi - 2*qf + 2*T*dqf))))/2 - 1)*((dqf - dqi)/(dqf*dt - dqi*dt) - (dqf - dqi)/(((dqf*dt - dqi*dt)/(2*qi - 2*qf + 2*T*dqf) - 2)*(2*qi - 2*qf + 2*T*dqf))) - (2^(1/2)*(log(2 - (dqf*dt - dqi*dt)/(2*qi - 2*qf + 2*T*dqf)) - log((dqf*dt - dqi*dt)/(2*qi - 2*qf + 2*T*dqf)))*((dqf - dqi)/(dqf*dt - dqi*dt) + (dqf - dqi)/(((dqf*dt - dqi*dt)/(2*qi - 2*qf + 2*T*dqf) - 2)*(2*qi - 2*qf + 2*T*dqf))))/2)^2*(tanh((log(2 - (dqf*dt - dqi*dt)/(2*qi - 2*qf + 2*T*dqf)) - log((dqf*dt - dqi*dt)/(2*qi - 2*qf + 2*T*dqf)))*((2^(1/2)*(log(2 - (dqf*dt - dqi*dt)/(2*qi - 2*qf + 2*T*dqf)) + log((dqf*dt - dqi*dt)/(2*qi - 2*qf + 2*T*dqf))))/2 - 1))^2 - 1)) + ((2*log((dqf*dt - dqi*dt)/(2*qi - 2*qf + 2*T*dqf))*(dqf - dqi))/(3*(dqf*dt - dqi*dt)) - (2*log(1 - (dqf*dt - dqi*dt)/(2*qi - 2*qf + 2*T*dqf))*(dqf - dqi))/(3*((dqf*dt - dqi*dt)/(2*qi - 2*qf + 2*T*dqf) - 1)*(2*qi - 2*qf + 2*T*dqf)))*(tanh(log((dqf*dt - dqi*dt)/(2*qi - 2*qf + 2*T*dqf))^2/3 - log(1 - (dqf*dt - dqi*dt)/(2*qi - 2*qf + 2*T*dqf))^2/3)^2 - 1)*((((2^(1/2)*(log(2 - (dqf*dt - dqi*dt)/(2*qi - 2*qf + 2*T*dqf)) + log((dqf*dt - dqi*dt)/(2*qi - 2*qf + 2*T*dqf))))/2 - 1)*((dqf - dqi)/(dqf*dt - dqi*dt) - (dqf - dqi)/(((dqf*dt - dqi*dt)/(2*qi - 2*qf + 2*T*dqf) - 2)*(2*qi - 2*qf + 2*T*dqf))) - (2^(1/2)*(log(2 - (dqf*dt - dqi*dt)/(2*qi - 2*qf + 2*T*dqf)) - log((dqf*dt - dqi*dt)/(2*qi - 2*qf + 2*T*dqf)))*((dqf - dqi)/(dqf*dt - dqi*dt) + (dqf - dqi)/(((dqf*dt - dqi*dt)/(2*qi - 2*qf + 2*T*dqf) - 2)*(2*qi - 2*qf + 2*T*dqf))))/2)*(tanh((log(2 - (dqf*dt - dqi*dt)/(2*qi - 2*qf + 2*T*dqf)) - log((dqf*dt - dqi*dt)/(2*qi - 2*qf + 2*T*dqf)))*((2^(1/2)*(log(2 - (dqf*dt - dqi*dt)/(2*qi - 2*qf + 2*T*dqf)) + log((dqf*dt - dqi*dt)/(2*qi - 2*qf + 2*T*dqf))))/2 - 1))^2 - 1) - (2*(dqf - dqi))/(2*qi - 2*qf + 2*T*dqf)) + (tanh(((2^(1/2)*(log((dqf*dt - dqi*dt)/(2*qi - 2*qf + 2*T*dqf) + 1) + log(1 - (dqf*dt - dqi*dt)/(2*qi - 2*qf + 2*T*dqf))))/2 - 1)*(log((dqf*dt - dqi*dt)/(2*qi - 2*qf + 2*T*dqf) + 1) - log(1 - (dqf*dt - dqi*dt)/(2*qi - 2*qf + 2*T*dqf))))^2 - 1)*(tanh(log((dqf*dt - dqi*dt)/(2*qi - 2*qf + 2*T*dqf))^2/3 - log(1 - (dqf*dt - dqi*dt)/(2*qi - 2*qf + 2*T*dqf))^2/3)/2 - 1/2)*(2^(1/2)*((dqf - dqi)/(((dqf*dt - dqi*dt)/(2*qi - 2*qf + 2*T*dqf) - 1)*(2*qi - 2*qf + 2*T*dqf)) + (dqf - dqi)/(((dqf*dt - dqi*dt)/(2*qi - 2*qf + 2*T*dqf) + 1)*(2*qi - 2*qf + 2*T*dqf)))*((dqf - dqi)/(((dqf*dt - dqi*dt)/(2*qi - 2*qf + 2*T*dqf) - 1) ...
                *(2*qi - 2*qf + 2*T*dqf)) - (dqf - dqi)/(((dqf*dt - dqi*dt)/(2*qi - 2*qf + 2*T*dqf) + 1)*(2*qi - 2*qf + 2*T*dqf))) - ((2^(1/2)*(log((dqf*dt - dqi*dt)/(2*qi - 2*qf + 2*T*dqf) + 1) + log(1 - (dqf*dt - dqi*dt)/(2*qi - 2*qf + 2*T*dqf))))/2 - 1)*((dqf - dqi)^2/(((dqf*dt - dqi*dt)/(2*qi - 2*qf + 2*T*dqf) - 1)^2*(2*qi - 2*qf + 2*T*dqf)^2) - (dqf - dqi)^2/(((dqf*dt - dqi*dt)/(2*qi - 2*qf + 2*T*dqf) + 1)^2*(2*qi - 2*qf + 2*T*dqf)^2)) + (2^(1/2)*(log((dqf*dt - dqi*dt)/(2*qi - 2*qf + 2*T*dqf) + 1) - log(1 - (dqf*dt - dqi*dt)/(2*qi - 2*qf + 2*T*dqf)))*((dqf - dqi)^2/(((dqf*dt - dqi*dt)/(2*qi - 2*qf + 2*T*dqf) - 1)^2*(2*qi - 2*qf + 2*T*dqf)^2) + (dqf - dqi)^2/(((dqf*dt - dqi*dt)/(2*qi - 2*qf + 2*T*dqf) + 1)^2*(2*qi - 2*qf + 2*T*dqf)^2)))/2) + tanh(((2^(1/2)*(log((dqf*dt - dqi*dt)/(2*qi - 2*qf + 2*T*dqf) + 1) + log(1 - (dqf*dt - dqi*dt)/(2*qi - 2*qf + 2*T*dqf))))/2 - 1)*(log((dqf*dt - dqi*dt)/(2*qi - 2*qf + 2*T*dqf) + 1) - log(1 - (dqf*dt - dqi*dt)/(2*qi - 2*qf + 2*T*dqf))))*tanh(log((dqf*dt - dqi*dt)/(2*qi - 2*qf + 2*T*dqf))^2/3 - log(1 - (dqf*dt - dqi*dt)/(2*qi - 2*qf + 2*T*dqf))^2/3)*((2*log((dqf*dt - dqi*dt)/(2*qi - 2*qf + 2*T*dqf))*(dqf - dqi))/(3*(dqf*dt - dqi*dt)) - (2*log(1 - (dqf*dt - dqi*dt)/(2*qi - 2*qf + 2*T*dqf))*(dqf - dqi))/(3*((dqf*dt - dqi*dt)/(2*qi - 2*qf + 2*T*dqf) - 1)*(2*qi - 2*qf + 2*T*dqf)))^2*(tanh(log((dqf*dt - dqi*dt)/(2*qi - 2*qf + 2*T*dqf))^2/3 - log(1 - (dqf*dt - dqi*dt)/(2*qi - 2*qf + 2*T*dqf))^2/3)^2 - 1) - (tanh(((2^(1/2)*(log((dqf*dt - dqi*dt)/(2*qi - 2*qf + 2*T*dqf) + 1) + log(1 - (dqf*dt - dqi*dt)/(2*qi - 2*qf + 2*T*dqf))))/2 - 1)*(log((dqf*dt - dqi*dt)/(2*qi - 2*qf + 2*T*dqf) + 1) - log(1 - (dqf*dt - dqi*dt)/(2*qi - 2*qf + 2*T*dqf))))^2 - 1)*((2*log((dqf*dt - dqi*dt)/(2*qi - 2*qf + 2*T*dqf))*(dqf - dqi))/(3*(dqf*dt - dqi*dt)) - (2*log(1 - (dqf*dt - dqi*dt)/(2*qi - 2*qf + 2*T*dqf))*(dqf - dqi))/(3*((dqf*dt - dqi*dt)/(2*qi - 2*qf + 2*T*dqf) - 1)*(2*qi - 2*qf + 2*T*dqf)))*(tanh(log((dqf*dt - dqi*dt)/(2*qi - 2*qf + 2*T*dqf))^2/3 - log(1 - (dqf*dt - dqi*dt)/(2*qi - 2*qf + 2*T*dqf))^2/3)^2 - 1)*(((2^(1/2)*(log((dqf*dt - dqi*dt)/(2*qi - 2*qf + 2*T*dqf) + 1) + log(1 - (dqf*dt - dqi*dt)/(2*qi - 2*qf + 2*T*dqf))))/2 - 1)*((dqf - dqi)/(((dqf*dt - dqi*dt)/(2*qi - 2*qf + 2*T*dqf) - 1)*(2*qi - 2*qf + 2*T*dqf)) - (dqf - dqi)/(((dqf*dt - dqi*dt)/(2*qi - 2*qf + 2*T*dqf) + 1)*(2*qi - 2*qf + 2*T*dqf))) - (2^(1/2)*(log((dqf*dt - dqi*dt)/(2*qi - 2*qf + 2*T*dqf) + 1) - log(1 - (dqf*dt - dqi*dt)/(2*qi - 2*qf + 2*T*dqf)))*((dqf - dqi)/(((dqf*dt - dqi*dt)/(2*qi - 2*qf + 2*T*dqf) - 1)*(2*qi - 2*qf + 2*T*dqf)) + (dqf - dqi)/(((dqf*dt - dqi*dt)/(2*qi - 2*qf + 2*T*dqf) + 1)*(2*qi - 2*qf + 2*T*dqf))))/2) - tanh(log((dqf*dt - dqi*dt)/(2*qi - 2*qf + 2*T*dqf))^2/3 - log(1 - (dqf*dt - dqi*dt)/(2*qi - 2*qf + 2*T*dqf))^2/3)*((2*log((dqf*dt - dqi*dt)/(2*qi - 2*qf + 2*T*dqf))*(dqf - dqi))/(3*(dqf*dt - ...
                dqi*dt)) - (2*log(1 - (dqf*dt - dqi*dt)/(2*qi - 2*qf + 2*T*dqf))*(dqf - dqi))/(3*((dqf*dt - dqi*dt)/(2*qi - 2*qf + 2*T*dqf) - 1)*(2*qi - 2*qf + 2*T*dqf)))^2*(tanh(log((dqf*dt - dqi*dt)/(2*qi - 2*qf + 2*T*dqf))^2/3 - log(1 - (dqf*dt - dqi*dt)/(2*qi - 2*qf + 2*T*dqf))^2/3)^2 - 1)*(tanh((log(2 - (dqf*dt - dqi*dt)/(2*qi - 2*qf + 2*T*dqf)) - log((dqf*dt - dqi*dt)/(2*qi - 2*qf + 2*T*dqf)))*((2^(1/2)*(log(2 - (dqf*dt - dqi*dt)/(2*qi - 2*qf + 2*T*dqf)) + log((dqf*dt - dqi*dt)/(2*qi - 2*qf + 2*T*dqf))))/2 - 1)) - (2*(dqf*dt - dqi*dt))/(2*qi - 2*qf + 2*T*dqf) + 1) + 2*tanh(((2^(1/2)*(log((dqf*dt - dqi*dt)/(2*qi - 2*qf + 2*T*dqf) + 1) + log(1 - (dqf*dt - dqi*dt)/(2*qi - 2*qf + 2*T*dqf))))/2 - 1)*(log((dqf*dt - dqi*dt)/(2*qi - 2*qf + 2*T*dqf) + 1) - log(1 - (dqf*dt - dqi*dt)/(2*qi - 2*qf + 2*T*dqf))))*(tanh(((2^(1/2)*(log((dqf*dt - dqi*dt)/(2*qi - 2*qf + 2*T*dqf) + 1) + log(1 - (dqf*dt - dqi*dt)/(2*qi - 2*qf + 2*T*dqf))))/2 - 1)*(log((dqf*dt - dqi*dt)/(2*qi - 2*qf + 2*T*dqf) + 1) - log(1 - (dqf*dt - dqi*dt)/(2*qi - 2*qf + 2*T*dqf))))^2 - 1)*(tanh(log((dqf*dt - dqi*dt)/(2*qi - 2*qf + 2*T*dqf))^2/3 - log(1 - (dqf*dt - dqi*dt)/(2*qi - 2*qf + 2*T*dqf))^2/3)/2 - 1/2)*(((2^(1/2)*(log((dqf*dt - dqi*dt)/(2*qi - 2*qf + 2*T*dqf) + 1) + log(1 - (dqf*dt - dqi*dt)/(2*qi - 2*qf + 2*T*dqf))))/2 - 1)*((dqf - dqi)/(((dqf*dt - dqi*dt)/(2*qi - 2*qf + 2*T*dqf) - 1)*(2*qi - 2*qf + 2*T*dqf)) - (dqf - dqi)/(((dqf*dt - dqi*dt)/(2*qi - 2*qf + 2*T*dqf) + 1)*(2*qi - 2*qf + 2*T*dqf))) - (2^(1/2)*(log((dqf*dt - dqi*dt)/(2*qi - 2*qf + 2*T*dqf) + 1) - log(1 - (dqf*dt - dqi*dt)/(2*qi - 2*qf + 2*T*dqf)))*((dqf - dqi)/(((dqf*dt - dqi*dt)/(2*qi - 2*qf + 2*T*dqf) - 1)*(2*qi - 2*qf + 2*T*dqf)) + (dqf - dqi)/(((dqf*dt - dqi*dt)/(2*qi - 2*qf + 2*T*dqf) + 1)*(2*qi - 2*qf + 2*T*dqf))))/2)^2);

            qv = [qd;dqd;ddqd]; %Send values back
        else 
            qv = [0;0;0];
        end
    else
        qv = [0;0;0];
    end
end

end

function ris=compute_traj_parameters(s0, v0, sf, vm, am)
    ris=zeros(15,1);
    radix=zeros(2,1);
    T1 = 0;
    dT = 0;
    T2 = 0;
    a1 = 0;
    b1 = 0;
    c1 = 0;
    d1 = 0;
    e1 = 0;
    a2 = 0;
    b2 = 0;
    c2 = 0;
    d2 = 0;
    e2 = 0;
    k = 0;

    if (vm~=0) %check...
        vm=vm*sign(sf-s0);
        k=am*sign(sf-s0);
        T1 = -3/2*(v0-vm)/k;
        a1 = -4/27*k^3/(v0-vm)^2;
        b1 = -4/9*k^2/(v0-vm);
        e1 = s0;
        d1 = v0;
        c1 = 0;
        c2 = 0;
        T2 = 3/2*vm/k;
        dT = 1/4*(-3*vm^2+4*sf*k-4*a1*T1^4*k-4*b1*T1^3*k-4*c1*T1^2*k-4*d1*T1*k-4*e1*k)/vm/k;
        a2 = 4/27*k^3/vm^2;
        d2 = vm;
        e2 = 1/4*(-3*vm^2+4*sf*k)/k;
        b2 = -4/9*k^2/vm;
        if (dT<0)
            c2 = 0;
            c1 = 0;
            a=2;
            b=12*v0;
            c=9*v0^2-12*sf*k+12*s0*k;
            radix(1)=(-b + sqrt(b^2-4*a*c))/(2*a);
            radix(2)=(-b - sqrt(b^2-4*a*c))/(2*a);
            %decide the correct root
            T1_a = 1/2*radix(1)/k;
            T2_a = 1/2*(radix(1)+3*v0)/k;
            T1_b = 1/2*radix(2)/k;
            T2_b = 1/2*(radix(2)+3*v0)/k;
                if (and(T1_a>=0, T2_a>=0))
                    r=radix(1);
                    T1=T1_a;
                    T2=T2_a;
                    dT=0;
                    two_phases=1;
                elseif (and(T1_b>=0, T2_b>=0))
                    r=radix(2);
                    T1=T1_b;
                    T2=T2_b;
                    dT=0;
                    two_phases=1;
                else
                    r=0;
                    two_phases=0;
                end
                if (two_phases==0)
                    T1=0;
                    T2=2*(sf-s0)/v0;
                    dT=0;
                    b2=-1/4*v0^3/(sf-s0)^2;
                    c2=0;
                    a2=1/16*v0^4/(sf-s0)^3;
                    d2=v0;
                    e2=s0;
                else
                    b1 = -8/9*k^2/(4*v0*r+3*v0^2-4*sf*k+4*s0*k)*r;
                    a1 = 8/9*k^3/(4*v0*r+3*v0^2-4*sf*k+4*s0*k);
                    b2 = -8/9*k^2/(4*sf*k+3*v0^2-4*s0*k)*(r+3*v0);
                    e2 = -1/8*(3*v0^2-4*s0*k-4*sf*k)/k;
                    e1 = s0;
                    d1 = v0;
                    d2 = 2/9/(4*sf*k+3*v0^2-4*s0*k)*(r+3*v0)^3;
                    a2 = 8/9*k^3/(4*sf*k+3*v0^2-4*s0*k);
                end
        end
    end
    ris=[T1;dT;T2; a1; b1; c1; d1; e1; a2; b2; c2; d2; e2; vm; k];
end

%time, and the output of the previous function
function [ris, finished]=interpolator(t, parameters)

ris=zeros(3,1);
T1=parameters(1);
dT=parameters(2);
T2=parameters(3);
a1=parameters(4);
b1=parameters(5);
c1=parameters(6);
d1=parameters(7);
e1=parameters(8);
a2=parameters(9);
b2=parameters(10);
c2=parameters(11);
d2=parameters(12);
e2=parameters(13);
vm=parameters(14);
k=parameters(15);

finished = 0;
if (vm~=0) %check...
        if (t<=T1)
            ris=[a1*t^4+b1*t^3+c1*t^2+d1*t+e1; 4*a1*t^3+3*b1*t^2+2*c1*t+d1; 12*a1*t^2+6*b1*t+2*c1];
        elseif (t<=T1+dT)
            t=t-T1;
            ris=[a1*T1^4+b1*T1^3+c1*T1^2+d1*T1+e1+vm*t; vm; 0];
        elseif (t<=T1+dT+T2)
            t=t-T1-dT;
            ris=[a2*t^4+b2*t^3+c2*t^2+d2*t+e2; 4*a2*t^3+3*b2*t^2+2*c2*t+d2; 12*a2*t^2+6*b2*t+2*c2];
        else
            t=T2;
            ris=[a2*t^4+b2*t^3+c2*t^2+d2*t+e2;0;0];
            finished=1;
        end
else
    ris=[0;0;0];
end

end

function t=interpolator_1(q, parameters)

T1=parameters(1);
dT=parameters(2);
T2=parameters(3);
a1=parameters(4);
b1=parameters(5);
c1=parameters(6);
d1=parameters(7);
e1=parameters(8);
a2=parameters(9);
b2=parameters(10);
c2=parameters(11);
d2=parameters(12);
e2=parameters(13);
vm=parameters(14);
k=parameters(15);

t=0;
Q1 = a1*T1^4+b1*T1^3+c1*T1^2+d1*T1+e1;%q point at end of startup
Q2 = a2*T2^4+b2*T2^3+c2*T2^2+d2*T2+e2;%final q
Q3 = Q2-Q1;%q point at end of linear part (using symmetry)

if q<Q1
    %startup
%     %tarray = 0:0.001:T1; %not working, because T1 should be constant?!
%     tarray = linspace(0,T1);
%     qarray=zeros(size(tarray));
%     parfor i=1:size(tarray,2)
%         [qv,~]=interpolator(tarray(i), parameters);
%         qarray(i)=qv(1);
%     end
%     t = interp1(qarray, tarray, q);
    t=0;
    %error('trans: interpolator_1 startup: not programmed jet, sry');
    % problem with calculating additional shift
elseif q>=Q1 && q<=Q3
    %linear part
    t = T1+((q-Q1)/vm);
elseif q>Q3
    %slowdown
    t=-1;
    %error('trans: interpolator_1 slowdown: not programmed jet, sry');
end

end
